simulink model "Copter_Plane_h2g_4_and_1"  (R2020a)
settings: Solver=ode1  StartTime=0.0  StopTime=100  FixedStep=dt  RelTol=1e-3
(part 1 of 2)
settings Model: xpc_rtwmakecfg_data=_xpcnblib_  PauseTimes=2  Creator=a4327  LastModifiedBy=a4327
settings DataIOCC: ReturnWorkspaceOutputs=off
settings OptimizationCC: DefaultParameterBehavior=Inlined  UseDivisionForNetSlopeComputation=on  GainParamInheritBuiltInType=on  UseFloatMulNetSlope=on  InlineInvariantSignals=on  PassReuseOutputArgsAs=Individual arguments  ZeroExternalMemoryAtStartup=off  ZeroInternalMemoryAtStartup=off  NoFixptDivByZeroProtection=on  EfficientFloat2IntCast=on  LifeSpan=1  OptimizeBlockOrder=speed  DifferentSizesBufferReuse=on  EfficientTunableParamExpr=on
settings DebuggingCC: ParameterTunabilityLossMsg=error  ArithmeticOperatorsInVariantConditions=warning
settings HardwareCC: ProdBitPerPointer=32  ProdBitPerSizeT=32  ProdBitPerPtrDiffT=32  ProdLargestAtomicFloat=None  ProdWordSize=32  ProdLongLongMode=on  ProdHWDeviceType=Custom Processor->Custom Processor
settings SFSimCC: MATLABDynamicMemAlloc=off  CustomCodeUndefinedFunction=UseInterfaceOnly
settings RTWCC: SystemTargetFile=ert.tlc  TemplateMakefile=ert_default_tmf  GenerateReport=on  IncludeHyperlinkInReport=on  LaunchReport=on  GenerateTraceInfo=on  GenerateTraceReport=on  GenerateTraceReportSl=on  GenerateTraceReportSf=on  GenerateTraceReportEml=on  GenerateCodeMetricsReport=on
settings CodeAppCC: ForceParamTrailComments=on  IgnoreCustomStorageClasses=off  OperatorAnnotations=on  SimulinkDataObjDesc=on  SFDataObjDesc=on  CustomSymbolStrGlobalVar=rt$N$M  CustomSymbolStrType=$N$M  CustomSymbolStrFcn=$N$M$F  CustomSymbolStrMacro=$N$M  InsertBlockDesc=on
settings ERTTargetCC: TargetLangStandard=C99 (ISO)  GenerateSampleERTMain=on  IncludeMdlTerminateFcn=off  CombineSignalStateStructs=on  MultiInstanceERTCode=on  CodeInterfacePackaging=Reusable function  SupportComplex=off  SupportNonInlinedSFcns=on  InlinedParameterPlacement=NonHierarchical  RootIOFormat=Structure reference  ERTCustomFileTemplate=example_file_process.tlc  ERTFilePackagingFormat=CompactWithDataFile

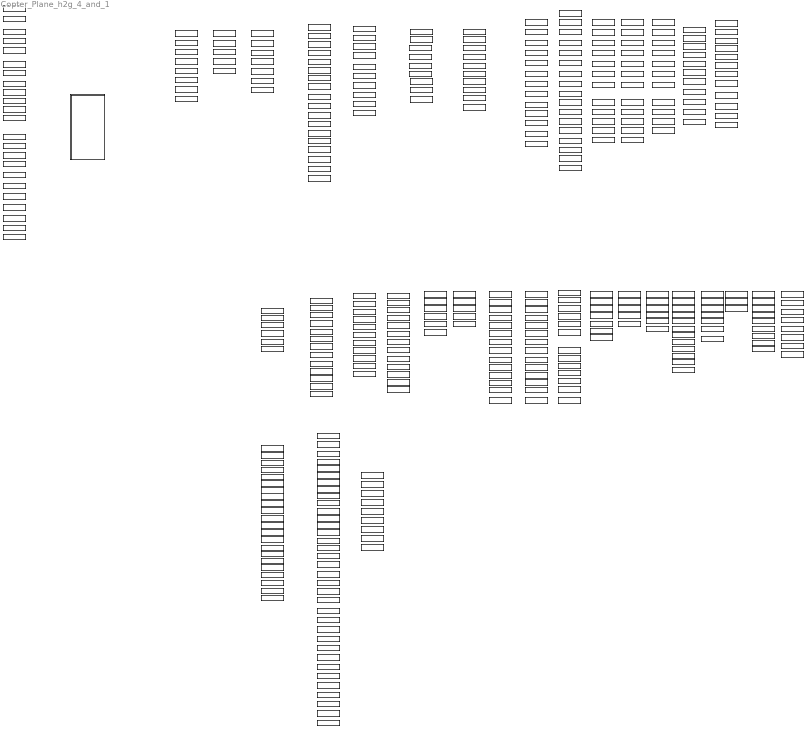
== system Copter_Plane_h2g_4_and_1 ==
  AC_ATTITUDE_ACCEL_RP_CONTROLLER_MAX_RADSS1 : DataStoreMemory  DataStoreName=AC_ATTITUDE_ACCEL_RP_CONTROLLER_MAX_RADSS  ReadBeforeWriteMsg=warning  WriteAfterWriteMsg=warning  WriteAfterReadMsg=warning  InitialValue=AC_ATTITUDE_ACCEL_RP_CONTROLLER_MAX_RADSS  VectorParams1D=off  ShowAdditionalParam=off  OutDataTypeStr=double
  AC_ATTITUDE_ACCEL_RP_CONTROLLER_MIN_RADSS1 : DataStoreMemory  DataStoreName=AC_ATTITUDE_ACCEL_RP_CONTROLLER_MIN_RADSS  ReadBeforeWriteMsg=warning  WriteAfterWriteMsg=warning  WriteAfterReadMsg=warning  InitialValue=AC_ATTITUDE_ACCEL_RP_CONTROLLER_MIN_RADSS  VectorParams1D=off  ShowAdditionalParam=off  OutDataTypeStr=double
  AC_ATTITUDE_ACCEL_Y_CONTROLLER_MAX_RADSS1 : DataStoreMemory  DataStoreName=AC_ATTITUDE_ACCEL_Y_CONTROLLER_MAX_RADSS  ReadBeforeWriteMsg=warning  WriteAfterWriteMsg=warning  WriteAfterReadMsg=warning  InitialValue=AC_ATTITUDE_ACCEL_Y_CONTROLLER_MAX_RADSS  ShowAdditionalParam=off  OutDataTypeStr=double
  AC_ATTITUDE_ACCEL_Y_CONTROLLER_MIN_RADSS1 : DataStoreMemory  DataStoreName=AC_ATTITUDE_ACCEL_Y_CONTROLLER_MIN_RADSS  ReadBeforeWriteMsg=warning  WriteAfterWriteMsg=warning  WriteAfterReadMsg=warning  InitialValue=AC_ATTITUDE_ACCEL_Y_CONTROLLER_MIN_RADSS  VectorParams1D=off  ShowAdditionalParam=off  OutDataTypeStr=double
  AC_ATTITUDE_CONTROL_ANGLE_LIMIT_THROTTLE_MAX1 : DataStoreMemory  DataStoreName=AC_ATTITUDE_CONTROL_ANGLE_LIMIT_THROTTLE_MAX  ReadBeforeWriteMsg=warning  WriteAfterWriteMsg=warning  WriteAfterReadMsg=warning  InitialValue=AC_ATTITUDE_CONTROL_ANGLE_LIMIT_THROTTLE_MAX  VectorParams1D=off  ShowAdditionalParam=off  OutDataTypeStr=double
  AC_ATTITUDE_CONTROL_MAX1 : DataStoreMemory  DataStoreName=AC_ATTITUDE_CONTROL_MAX  ReadBeforeWriteMsg=warning  WriteAfterWriteMsg=warning  WriteAfterReadMsg=warning  InitialValue=AC_ATTITUDE_CONTROL_MAX  VectorParams1D=off  ShowAdditionalParam=off  OutDataTypeStr=double
  AC_ATTITUDE_THRUST_ERROR_ANGLE1 : DataStoreMemory  DataStoreName=AC_ATTITUDE_THRUST_ERROR_ANGLE  ReadBeforeWriteMsg=warning  WriteAfterWriteMsg=warning  WriteAfterReadMsg=warning  InitialValue=AC_ATTITUDE_THRUST_ERROR_ANGLE  ShowAdditionalParam=off  OutDataTypeStr=double
  AP_MOTORS_MATRIX_YAW_FACTOR_CCW1 : DataStoreMemory  DataStoreName=AP_MOTORS_MATRIX_YAW_FACTOR_CCW  ReadBeforeWriteMsg=warning  WriteAfterWriteMsg=warning  WriteAfterReadMsg=warning  InitialValue=AP_MOTORS_MATRIX_YAW_FACTOR_CCW  VectorParams1D=off  ShowAdditionalParam=off  OutDataTypeStr=double
  AP_MOTORS_MATRIX_YAW_FACTOR_CW1 : DataStoreMemory  DataStoreName=AP_MOTORS_MATRIX_YAW_FACTOR_CW  ReadBeforeWriteMsg=warning  WriteAfterWriteMsg=warning  WriteAfterReadMsg=warning  InitialValue=AP_MOTORS_MATRIX_YAW_FACTOR_CW  VectorParams1D=off  ShowAdditionalParam=off  OutDataTypeStr=double
  ATC_RAT_PIT_D1 : DataStoreMemory  DataStoreName=ATC_RAT_PIT_D  ReadBeforeWriteMsg=warning  WriteAfterWriteMsg=warning  WriteAfterReadMsg=warning  InitialValue=ATC_RAT_PIT_D  VectorParams1D=off  ShowAdditionalParam=off  OutDataTypeStr=double
  ATC_RAT_PIT_FF1 : DataStoreMemory  DataStoreName=ATC_RAT_PIT_FF  ReadBeforeWriteMsg=warning  WriteAfterWriteMsg=warning  WriteAfterReadMsg=warning  InitialValue=ATC_RAT_PIT_FF  VectorParams1D=off  ShowAdditionalParam=off  OutDataTypeStr=double
  ATC_RAT_PIT_FILT1 : DataStoreMemory  DataStoreName=ATC_RAT_PIT_FILT  ReadBeforeWriteMsg=warning  WriteAfterWriteMsg=warning  WriteAfterReadMsg=warning  InitialValue=ATC_RAT_PIT_FILT  VectorParams1D=off  ShowAdditionalParam=off  OutDataTypeStr=double
  ATC_RAT_PIT_I1 : DataStoreMemory  DataStoreName=ATC_RAT_PIT_I  ReadBeforeWriteMsg=warning  WriteAfterWriteMsg=warning  WriteAfterReadMsg=warning  InitialValue=ATC_RAT_PIT_I  VectorParams1D=off  ShowAdditionalParam=off  OutDataTypeStr=double
  ATC_RAT_PIT_IMAX1 : DataStoreMemory  DataStoreName=ATC_RAT_PIT_IMAX  ReadBeforeWriteMsg=warning  WriteAfterWriteMsg=warning  WriteAfterReadMsg=warning  InitialValue=ATC_RAT_PIT_IMAX  VectorParams1D=off  ShowAdditionalParam=off  OutDataTypeStr=double
  ATC_RAT_PIT_I_inint1 : DataStoreMemory  DataStoreName=ATC_RAT_PIT_I_inint  ReadBeforeWriteMsg=warning  WriteAfterWriteMsg=warning  WriteAfterReadMsg=warning  InitialValue=ATC_RAT_PIT_I_inint  VectorParams1D=off  ShowAdditionalParam=off  OutDataTypeStr=double
  ATC_RAT_PIT_P1 : DataStoreMemory  DataStoreName=ATC_RAT_PIT_P  ReadBeforeWriteMsg=warning  WriteAfterWriteMsg=warning  WriteAfterReadMsg=warning  InitialValue=ATC_RAT_PIT_P  VectorParams1D=off  ShowAdditionalParam=off  OutDataTypeStr=double
  ATC_RAT_RLL_D1 : DataStoreMemory  DataStoreName=ATC_RAT_RLL_D  ReadBeforeWriteMsg=warning  WriteAfterWriteMsg=warning  WriteAfterReadMsg=warning  InitialValue=ATC_RAT_RLL_D  VectorParams1D=off  ShowAdditionalParam=off  OutDataTypeStr=double
  ATC_RAT_RLL_FF1 : DataStoreMemory  DataStoreName=ATC_RAT_RLL_FF  ReadBeforeWriteMsg=warning  WriteAfterWriteMsg=warning  WriteAfterReadMsg=warning  InitialValue=ATC_RAT_RLL_FF  VectorParams1D=off  ShowAdditionalParam=off  OutDataTypeStr=double
  ATC_RAT_RLL_FILT1 : DataStoreMemory  DataStoreName=ATC_RAT_RLL_FILT  ReadBeforeWriteMsg=warning  WriteAfterWriteMsg=warning  WriteAfterReadMsg=warning  InitialValue=ATC_RAT_RLL_FILT  VectorParams1D=off  ShowAdditionalParam=off  OutDataTypeStr=double
  ATC_RAT_RLL_I1 : DataStoreMemory  DataStoreName=ATC_RAT_RLL_I  ReadBeforeWriteMsg=warning  WriteAfterWriteMsg=warning  WriteAfterReadMsg=warning  InitialValue=ATC_RAT_RLL_I  VectorParams1D=off  ShowAdditionalParam=off  OutDataTypeStr=double
  ATC_RAT_RLL_IMAX1 : DataStoreMemory  DataStoreName=ATC_RAT_RLL_IMAX  ReadBeforeWriteMsg=warning  WriteAfterWriteMsg=warning  WriteAfterReadMsg=warning  InitialValue=ATC_RAT_RLL_IMAX  VectorParams1D=off  ShowAdditionalParam=off  OutDataTypeStr=double
  ATC_RAT_RLL_I_inint1 : DataStoreMemory  DataStoreName=ATC_RAT_RLL_I_inint  ReadBeforeWriteMsg=warning  WriteAfterWriteMsg=warning  WriteAfterReadMsg=warning  InitialValue=ATC_RAT_RLL_I_inint  VectorParams1D=off  ShowAdditionalParam=off  OutDataTypeStr=double
  ATC_RAT_RLL_P1 : DataStoreMemory  DataStoreName=ATC_RAT_RLL_P  ReadBeforeWriteMsg=warning  WriteAfterWriteMsg=warning  WriteAfterReadMsg=warning  InitialValue=ATC_RAT_RLL_P  VectorParams1D=off  ShowAdditionalParam=off  OutDataTypeStr=double
  ATC_RAT_YAW_D1 : DataStoreMemory  DataStoreName=ATC_RAT_YAW_D  ReadBeforeWriteMsg=warning  WriteAfterWriteMsg=warning  WriteAfterReadMsg=warning  InitialValue=ATC_RAT_YAW_D  VectorParams1D=off  ShowAdditionalParam=off  OutDataTypeStr=double
  ATC_RAT_YAW_FF1 : DataStoreMemory  DataStoreName=ATC_RAT_YAW_FF  ReadBeforeWriteMsg=warning  WriteAfterWriteMsg=warning  WriteAfterReadMsg=warning  InitialValue=ATC_RAT_YAW_FF  VectorParams1D=off  ShowAdditionalParam=off  OutDataTypeStr=double
  ATC_RAT_YAW_FILT1 : DataStoreMemory  DataStoreName=ATC_RAT_YAW_FILT  ReadBeforeWriteMsg=warning  WriteAfterWriteMsg=warning  WriteAfterReadMsg=warning  InitialValue=ATC_RAT_YAW_FILT  VectorParams1D=off  ShowAdditionalParam=off  OutDataTypeStr=double
  ATC_RAT_YAW_I1 : DataStoreMemory  DataStoreName=ATC_RAT_YAW_I  ReadBeforeWriteMsg=warning  WriteAfterWriteMsg=warning  WriteAfterReadMsg=warning  InitialValue=ATC_RAT_YAW_I  VectorParams1D=off  ShowAdditionalParam=off  OutDataTypeStr=double
  ATC_RAT_YAW_IMAX1 : DataStoreMemory  DataStoreName=ATC_RAT_YAW_IMAX  ReadBeforeWriteMsg=warning  WriteAfterWriteMsg=warning  WriteAfterReadMsg=warning  InitialValue=ATC_RAT_YAW_IMAX  VectorParams1D=off  ShowAdditionalParam=off  OutDataTypeStr=double
  ATC_RAT_YAW_I_inint1 : DataStoreMemory  DataStoreName=ATC_RAT_YAW_I_inint  ReadBeforeWriteMsg=warning  WriteAfterWriteMsg=warning  WriteAfterReadMsg=warning  InitialValue=ATC_RAT_YAW_I_inint  VectorParams1D=off  ShowAdditionalParam=off  OutDataTypeStr=double
  ATC_RAT_YAW_P1 : DataStoreMemory  DataStoreName=ATC_RAT_YAW_P  ReadBeforeWriteMsg=warning  WriteAfterWriteMsg=warning  WriteAfterReadMsg=warning  InitialValue=ATC_RAT_YAW_P  VectorParams1D=off  ShowAdditionalParam=off  OutDataTypeStr=double
  EAS2TAS1 : DataStoreMemory  DataStoreName=EAS2TAS  ReadBeforeWriteMsg=warning  WriteAfterWriteMsg=warning  WriteAfterReadMsg=warning  InitialValue=EAS2TAS  VectorParams1D=off  ShowAdditionalParam=off  OutDataTypeStr=double
  EAS_dem1 : DataStoreMemory  DataStoreName=EAS_dem  ReadBeforeWriteMsg=warning  WriteAfterWriteMsg=warning  WriteAfterReadMsg=warning  InitialValue=EAS_dem  VectorParams1D=off  ShowAdditionalParam=off  OutDataTypeStr=double
  EAS_dem_cm1 : DataStoreMemory  DataStoreName=EAS_dem_cm  ReadBeforeWriteMsg=warning  WriteAfterWriteMsg=warning  WriteAfterReadMsg=warning  InitialValue=EAS_dem_cm  VectorParams1D=off  ShowAdditionalParam=off  OutDataTypeStr=double
  GRAVITY_MSS1 : DataStoreMemory  DataStoreName=GRAVITY_MSS  ReadBeforeWriteMsg=warning  WriteAfterWriteMsg=warning  WriteAfterReadMsg=warning  InitialValue=GRAVITY_MSS  VectorParams1D=off  ShowAdditionalParam=off  OutDataTypeStr=double
  HD1 : DataStoreMemory  DataStoreName=HD  ReadBeforeWriteMsg=warning  WriteAfterWriteMsg=warning  WriteAfterReadMsg=warning  InitialValue=HD  ShowAdditionalParam=off  OutDataTypeStr=double
  K_A_yaw1 : DataStoreMemory  DataStoreName=K_A_yaw  ReadBeforeWriteMsg=warning  WriteAfterWriteMsg=warning  WriteAfterReadMsg=warning  InitialValue=K_A_yaw  ShowAdditionalParam=off  OutDataTypeStr=double
  K_D_last_yaw1 : DataStoreMemory  DataStoreName=K_D_last_yaw  ReadBeforeWriteMsg=warning  WriteAfterWriteMsg=warning  WriteAfterReadMsg=warning  InitialValue=K_D_last_yaw  ShowAdditionalParam=off  OutDataTypeStr=double
  K_D_yaw1 : DataStoreMemory  DataStoreName=K_D_yaw  ReadBeforeWriteMsg=warning  WriteAfterWriteMsg=warning  WriteAfterReadMsg=warning  InitialValue=K_D_yaw  ShowAdditionalParam=off  OutDataTypeStr=double
  K_FF_yaw1 : DataStoreMemory  DataStoreName=K_FF_yaw  ReadBeforeWriteMsg=warning  WriteAfterWriteMsg=warning  WriteAfterReadMsg=warning  InitialValue=K_FF_yaw  ShowAdditionalParam=off  OutDataTypeStr=double
  K_FF_yaw_inint1 : DataStoreMemory  DataStoreName=K_FF_yaw_inint  ReadBeforeWriteMsg=warning  WriteAfterWriteMsg=warning  WriteAfterReadMsg=warning  InitialValue=K_FF_yaw_inint  VectorParams1D=off  ShowAdditionalParam=off  OutDataTypeStr=double
  K_I_yaw1 : DataStoreMemory  DataStoreName=K_I_yaw  ReadBeforeWriteMsg=warning  WriteAfterWriteMsg=warning  WriteAfterReadMsg=warning  InitialValue=K_I_yaw  ShowAdditionalParam=off  OutDataTypeStr=double
  Kx1 : DataStoreMemory  DataStoreName=Kx  ReadBeforeWriteMsg=warning  WriteAfterWriteMsg=warning  WriteAfterReadMsg=warning  InitialValue=Kx  VectorParams1D=off  ShowAdditionalParam=off  OutDataTypeStr=double
  L1_damping1 : DataStoreMemory  DataStoreName=L1_damping  ReadBeforeWriteMsg=warning  WriteAfterWriteMsg=warning  WriteAfterReadMsg=warning  InitialValue=L1_damping  VectorParams1D=off  ShowAdditionalParam=off  OutDataTypeStr=double
  L1_dist1 : DataStoreMemory  DataStoreName=L1_dist  ReadBeforeWriteMsg=warning  WriteAfterWriteMsg=warning  WriteAfterReadMsg=warning  InitialValue=L1_dist  VectorParams1D=off  ShowAdditionalParam=off  OutDataTypeStr=double
  L1_period1 : DataStoreMemory  DataStoreName=L1_period  ReadBeforeWriteMsg=warning  WriteAfterWriteMsg=warning  WriteAfterReadMsg=warning  InitialValue=L1_period  VectorParams1D=off  ShowAdditionalParam=off  OutDataTypeStr=double
  L1_radius1 : DataStoreMemory  DataStoreName=L1_radius  ReadBeforeWriteMsg=warning  WriteAfterWriteMsg=warning  WriteAfterReadMsg=warning  InitialValue=L1_radius  VectorParams1D=off  ShowAdditionalParam=off  OutDataTypeStr=double
  L1_xtrack_i1 : DataStoreMemory  DataStoreName=L1_xtrack_i  ReadBeforeWriteMsg=warning  WriteAfterWriteMsg=warning  WriteAfterReadMsg=warning  InitialValue=L1_xtrack_i  VectorParams1D=off  ShowAdditionalParam=off  OutDataTypeStr=double
  L1_xtrack_i_gain1 : DataStoreMemory  DataStoreName=L1_xtrack_i_gain  ReadBeforeWriteMsg=warning  WriteAfterWriteMsg=warning  WriteAfterReadMsg=warning  InitialValue=L1_xtrack_i_gain  VectorParams1D=off  ShowAdditionalParam=off  OutDataTypeStr=double
  L1_xtrack_i_gain_prev1 : DataStoreMemory  DataStoreName=L1_xtrack_i_gain_prev  ReadBeforeWriteMsg=warning  WriteAfterWriteMsg=warning  WriteAfterReadMsg=warning  InitialValue=L1_xtrack_i_gain_prev  VectorParams1D=off  ShowAdditionalParam=off  OutDataTypeStr=double
  LOCATION_SCALING_FACTOR1 : DataStoreMemory  DataStoreName=LOCATION_SCALING_FACTOR  ReadBeforeWriteMsg=warning  WriteAfterWriteMsg=warning  WriteAfterReadMsg=warning  InitialValue=LOCATION_SCALING_FACTOR  VectorParams1D=off  ShowAdditionalParam=off  OutDataTypeStr=double
  LOCATION_SCALING_FACTOR_INV1 : DataStoreMemory  DataStoreName=LOCATION_SCALING_FACTOR_INV  ReadBeforeWriteMsg=warning  WriteAfterWriteMsg=warning  WriteAfterReadMsg=warning  InitialValue=LOCATION_SCALING_FACTOR_INV  VectorParams1D=off  ShowAdditionalParam=off  OutDataTypeStr=double
  PITCHmaxf1 : DataStoreMemory  DataStoreName=PITCHmaxf  ReadBeforeWriteMsg=warning  WriteAfterWriteMsg=warning  WriteAfterReadMsg=warning  InitialValue=PITCHmaxf  VectorParams1D=off  ShowAdditionalParam=off  OutDataTypeStr=double
  PITCHminf1 : DataStoreMemory  DataStoreName=PITCHminf  ReadBeforeWriteMsg=warning  WriteAfterWriteMsg=warning  WriteAfterReadMsg=warning  InitialValue=PITCHminf  VectorParams1D=off  ShowAdditionalParam=off  OutDataTypeStr=double
  POSCONTROL_ACCELERATION_MIN1 : DataStoreMemory  DataStoreName=POSCONTROL_ACCELERATION_MIN  ReadBeforeWriteMsg=warning  WriteAfterWriteMsg=warning  WriteAfterReadMsg=warning  InitialValue=POSCONTROL_ACCELERATION_MIN  ShowAdditionalParam=off  OutDataTypeStr=double
  POSCONTROL_ACCEL_FILTER_HZ1 : DataStoreMemory  DataStoreName=POSCONTROL_ACCEL_FILTER_HZ  ReadBeforeWriteMsg=warning  WriteAfterWriteMsg=warning  WriteAfterReadMsg=warning  InitialValue=POSCONTROL_ACCEL_FILTER_HZ  VectorParams1D=off  ShowAdditionalParam=off  OutDataTypeStr=double
  POSCONTROL_ACCEL_XY1 : DataStoreMemory  DataStoreName=POSCONTROL_ACCEL_XY  ReadBeforeWriteMsg=warning  WriteAfterWriteMsg=warning  WriteAfterReadMsg=warning  InitialValue=POSCONTROL_ACCEL_XY  VectorParams1D=off  ShowAdditionalParam=off  OutDataTypeStr=double
  POSCONTROL_ACCEL_XY_MAX1 : DataStoreMemory  DataStoreName=POSCONTROL_ACCEL_XY_MAX  ReadBeforeWriteMsg=warning  WriteAfterWriteMsg=warning  WriteAfterReadMsg=warning  InitialValue=POSCONTROL_ACCEL_XY_MAX  VectorParams1D=off  ShowAdditionalParam=off  OutDataTypeStr=double
  POSCONTROL_ACCEL_Z1 : DataStoreMemory  DataStoreName=POSCONTROL_ACCEL_Z  ReadBeforeWriteMsg=warning  WriteAfterWriteMsg=warning  WriteAfterReadMsg=warning  InitialValue=POSCONTROL_ACCEL_Z  ShowAdditionalParam=off  OutDataTypeStr=double
  POSCONTROL_ACC_Z_D1 : DataStoreMemory  DataStoreName=POSCONTROL_ACC_Z_D  ReadBeforeWriteMsg=warning  WriteAfterWriteMsg=warning  WriteAfterReadMsg=warning  InitialValue=POSCONTROL_ACC_Z_D  VectorParams1D=off  ShowAdditionalParam=off  OutDataTypeStr=double
  POSCONTROL_ACC_Z_FILT_HZ1 : DataStoreMemory  DataStoreName=POSCONTROL_ACC_Z_FILT_HZ  ReadBeforeWriteMsg=warning  WriteAfterWriteMsg=warning  WriteAfterReadMsg=warning  InitialValue=POSCONTROL_ACC_Z_FILT_HZ  VectorParams1D=off  ShowAdditionalParam=off  OutDataTypeStr=double
  POSCONTROL_ACC_Z_FILT_HZ_c2p1 : DataStoreMemory  DataStoreName=POSCONTROL_ACC_Z_FILT_HZ_c2p  ReadBeforeWriteMsg=warning  WriteAfterWriteMsg=warning  WriteAfterReadMsg=warning  InitialValue=POSCONTROL_ACC_Z_FILT_HZ_c2p  VectorParams1D=off  ShowAdditionalParam=off  OutDataTypeStr=double
  POSCONTROL_ACC_Z_FILT_HZ_inint1 : DataStoreMemory  DataStoreName=POSCONTROL_ACC_Z_FILT_HZ_inint  ReadBeforeWriteMsg=warning  WriteAfterWriteMsg=warning  WriteAfterReadMsg=warning  InitialValue=POSCONTROL_ACC_Z_FILT_HZ_inint  VectorParams1D=off  ShowAdditionalParam=off  OutDataTypeStr=double
  POSCONTROL_ACC_Z_I1 : DataStoreMemory  DataStoreName=POSCONTROL_ACC_Z_I  ReadBeforeWriteMsg=warning  WriteAfterWriteMsg=warning  WriteAfterReadMsg=warning  InitialValue=POSCONTROL_ACC_Z_I  VectorParams1D=off  ShowAdditionalParam=off  OutDataTypeStr=double
  POSCONTROL_ACC_Z_IMAX1 : DataStoreMemory  DataStoreName=POSCONTROL_ACC_Z_IMAX  ReadBeforeWriteMsg=warning  WriteAfterWriteMsg=warning  WriteAfterReadMsg=warning  InitialValue=POSCONTROL_ACC_Z_IMAX  VectorParams1D=off  ShowAdditionalParam=off  OutDataTypeStr=double
  POSCONTROL_ACC_Z_I_inint1 : DataStoreMemory  DataStoreName=POSCONTROL_ACC_Z_I_inint  ReadBeforeWriteMsg=warning  WriteAfterWriteMsg=warning  WriteAfterReadMsg=warning  InitialValue=POSCONTROL_ACC_Z_I_inint  VectorParams1D=off  ShowAdditionalParam=off  OutDataTypeStr=double
  POSCONTROL_ACC_Z_P1 : DataStoreMemory  DataStoreName=POSCONTROL_ACC_Z_P  ReadBeforeWriteMsg=warning  WriteAfterWriteMsg=warning  WriteAfterReadMsg=warning  InitialValue=POSCONTROL_ACC_Z_P  VectorParams1D=off  ShowAdditionalParam=off  OutDataTypeStr=double
  POSCONTROL_JERK_RATIO1 : DataStoreMemory  DataStoreName=POSCONTROL_JERK_RATIO  ReadBeforeWriteMsg=warning  WriteAfterWriteMsg=warning  WriteAfterReadMsg=warning  InitialValue=POSCONTROL_JERK_RATIO  VectorParams1D=off  ShowAdditionalParam=off  OutDataTypeStr=double
  POSCONTROL_LEASH_LENGTH_MIN1 : DataStoreMemory  DataStoreName=POSCONTROL_LEASH_LENGTH_MIN  ReadBeforeWriteMsg=warning  WriteAfterWriteMsg=warning  WriteAfterReadMsg=warning  InitialValue=POSCONTROL_LEASH_LENGTH_MIN  VectorParams1D=off  ShowAdditionalParam=off  OutDataTypeStr=double
  POSCONTROL_OVERSPEED_GAIN_Z1 : DataStoreMemory  DataStoreName=POSCONTROL_OVERSPEED_GAIN_Z  ReadBeforeWriteMsg=warning  WriteAfterWriteMsg=warning  WriteAfterReadMsg=warning  InitialValue=POSCONTROL_OVERSPEED_GAIN_Z  VectorParams1D=off  ShowAdditionalParam=off  OutDataTypeStr=double
  POSCONTROL_POS_XY_P1 : DataStoreMemory  DataStoreName=POSCONTROL_POS_XY_P  ReadBeforeWriteMsg=warning  WriteAfterWriteMsg=warning  WriteAfterReadMsg=warning  InitialValue=POSCONTROL_POS_XY_P  VectorParams1D=off  ShowAdditionalParam=off  OutDataTypeStr=double
  POSCONTROL_POS_Z_P1 : DataStoreMemory  DataStoreName=POSCONTROL_POS_Z_P  ReadBeforeWriteMsg=warning  WriteAfterWriteMsg=warning  WriteAfterReadMsg=warning  InitialValue=POSCONTROL_POS_Z_P  VectorParams1D=off  ShowAdditionalParam=off  OutDataTypeStr=double
  POSCONTROL_SPEED1 : DataStoreMemory  DataStoreName=POSCONTROL_SPEED  ReadBeforeWriteMsg=warning  WriteAfterWriteMsg=warning  WriteAfterReadMsg=warning  InitialValue=POSCONTROL_SPEED  ShowAdditionalParam=off  OutDataTypeStr=double
  POSCONTROL_SPEED_DOWN1 : DataStoreMemory  DataStoreName=POSCONTROL_SPEED_DOWN  ReadBeforeWriteMsg=warning  WriteAfterWriteMsg=warning  WriteAfterReadMsg=warning  InitialValue=POSCONTROL_SPEED_DOWN  ShowAdditionalParam=off  OutDataTypeStr=double
  POSCONTROL_SPEED_UP1 : DataStoreMemory  DataStoreName=POSCONTROL_SPEED_UP  ReadBeforeWriteMsg=warning  WriteAfterWriteMsg=warning  WriteAfterReadMsg=warning  InitialValue=POSCONTROL_SPEED_UP  ShowAdditionalParam=off  OutDataTypeStr=double
  POSCONTROL_STOPPING_DIST_DOWN_MAX1 : DataStoreMemory  DataStoreName=POSCONTROL_STOPPING_DIST_DOWN_MAX  ReadBeforeWriteMsg=warning  WriteAfterWriteMsg=warning  WriteAfterReadMsg=warning  InitialValue=POSCONTROL_STOPPING_DIST_DOWN_MAX  VectorParams1D=off  ShowAdditionalParam=off  OutDataTypeStr=double
  POSCONTROL_STOPPING_DIST_UP_MAX1 : DataStoreMemory  DataStoreName=POSCONTROL_STOPPING_DIST_UP_MAX  ReadBeforeWriteMsg=warning  WriteAfterWriteMsg=warning  WriteAfterReadMsg=warning  InitialValue=POSCONTROL_STOPPING_DIST_UP_MAX  VectorParams1D=off  ShowAdditionalParam=off  OutDataTypeStr=double
  POSCONTROL_THROTTLE_CUTOFF_FREQ1 : DataStoreMemory  DataStoreName=POSCONTROL_THROTTLE_CUTOFF_FREQ  ReadBeforeWriteMsg=warning  WriteAfterWriteMsg=warning  WriteAfterReadMsg=warning  InitialValue=POSCONTROL_THROTTLE_CUTOFF_FREQ  VectorParams1D=off  ShowAdditionalParam=off  OutDataTypeStr=double
  POSCONTROL_VEL_ERROR_CUTOFF_FREQ1 : DataStoreMemory  DataStoreName=POSCONTROL_VEL_ERROR_CUTOFF_FREQ  ReadBeforeWriteMsg=warning  WriteAfterWriteMsg=warning  WriteAfterReadMsg=warning  InitialValue=POSCONTROL_VEL_ERROR_CUTOFF_FREQ  VectorParams1D=off  ShowAdditionalParam=off  OutDataTypeStr=double
  POSCONTROL_VEL_XY_D1 : DataStoreMemory  DataStoreName=POSCONTROL_VEL_XY_D  ReadBeforeWriteMsg=warning  WriteAfterWriteMsg=warning  WriteAfterReadMsg=warning  InitialValue=POSCONTROL_VEL_XY_D  VectorParams1D=off  ShowAdditionalParam=off  OutDataTypeStr=double
  POSCONTROL_VEL_XY_FILT_D_HZ1 : DataStoreMemory  DataStoreName=POSCONTROL_VEL_XY_FILT_D_HZ  ReadBeforeWriteMsg=warning  WriteAfterWriteMsg=warning  WriteAfterReadMsg=warning  InitialValue=POSCONTROL_VEL_XY_FILT_D_HZ  VectorParams1D=off  ShowAdditionalParam=off  OutDataTypeStr=double
  POSCONTROL_VEL_XY_FILT_HZ1 : DataStoreMemory  DataStoreName=POSCONTROL_VEL_XY_FILT_HZ  ReadBeforeWriteMsg=warning  WriteAfterWriteMsg=warning  WriteAfterReadMsg=warning  InitialValue=POSCONTROL_VEL_XY_FILT_HZ  VectorParams1D=off  ShowAdditionalParam=off  OutDataTypeStr=double
  POSCONTROL_VEL_XY_I1 : DataStoreMemory  DataStoreName=POSCONTROL_VEL_XY_I  ReadBeforeWriteMsg=warning  WriteAfterWriteMsg=warning  WriteAfterReadMsg=warning  InitialValue=POSCONTROL_VEL_XY_I  VectorParams1D=off  ShowAdditionalParam=off  OutDataTypeStr=double
  POSCONTROL_VEL_XY_IMAX1 : DataStoreMemory  DataStoreName=POSCONTROL_VEL_XY_IMAX  ReadBeforeWriteMsg=warning  WriteAfterWriteMsg=warning  WriteAfterReadMsg=warning  InitialValue=POSCONTROL_VEL_XY_IMAX  VectorParams1D=off  ShowAdditionalParam=off  OutDataTypeStr=double
  POSCONTROL_VEL_XY_I_inint1 : DataStoreMemory  DataStoreName=POSCONTROL_VEL_XY_I_inint  ReadBeforeWriteMsg=warning  WriteAfterWriteMsg=warning  WriteAfterReadMsg=warning  InitialValue=POSCONTROL_VEL_XY_I_inint  VectorParams1D=off  ShowAdditionalParam=off  OutDataTypeStr=double
  POSCONTROL_VEL_XY_P1 : DataStoreMemory  DataStoreName=POSCONTROL_VEL_XY_P  ReadBeforeWriteMsg=warning  WriteAfterWriteMsg=warning  WriteAfterReadMsg=warning  InitialValue=POSCONTROL_VEL_XY_P  VectorParams1D=off  ShowAdditionalParam=off  OutDataTypeStr=double
  POSCONTROL_VEL_Z_P1 : DataStoreMemory  DataStoreName=POSCONTROL_VEL_Z_P  ReadBeforeWriteMsg=warning  WriteAfterWriteMsg=warning  WriteAfterReadMsg=warning  InitialValue=POSCONTROL_VEL_Z_P  VectorParams1D=off  ShowAdditionalParam=off  OutDataTypeStr=double
  PathModeOut1 : DataStoreMemory  DataStoreName=PathModeOut_sl  ReadBeforeWriteMsg=warning  WriteAfterWriteMsg=warning  WriteAfterReadMsg=warning  InitialValue=PathModeOut_sl  VectorParams1D=off  ShowAdditionalParam=off  OutDataTypeStr=Bus: BUS_TASK_PATH_OutParam
  SKE_dem1 : DataStoreMemory  DataStoreName=SKE_dem  ReadBeforeWriteMsg=warning  WriteAfterWriteMsg=warning  WriteAfterReadMsg=warning  InitialValue=SKE_dem  VectorParams1D=off  ShowAdditionalParam=off  OutDataTypeStr=double
  SKE_est1 : DataStoreMemory  DataStoreName=SKE_est  ReadBeforeWriteMsg=warning  WriteAfterWriteMsg=warning  WriteAfterReadMsg=warning  InitialValue=SKE_est  VectorParams1D=off  ShowAdditionalParam=off  OutDataTypeStr=double
  SKEdot1 : DataStoreMemory  DataStoreName=SKEdot  ReadBeforeWriteMsg=warning  WriteAfterWriteMsg=warning  WriteAfterReadMsg=warning  InitialValue=SKEdot  VectorParams1D=off  ShowAdditionalParam=off  OutDataTypeStr=double
  SKEdot_dem1 : DataStoreMemory  DataStoreName=SKEdot_dem  ReadBeforeWriteMsg=warning  WriteAfterWriteMsg=warning  WriteAfterReadMsg=warning  InitialValue=SKEdot_dem  VectorParams1D=off  ShowAdditionalParam=off  OutDataTypeStr=double
  SPE_dem1 : DataStoreMemory  DataStoreName=SPE_dem  ReadBeforeWriteMsg=warning  WriteAfterWriteMsg=warning  WriteAfterReadMsg=warning  InitialValue=SPE_dem  VectorParams1D=off  ShowAdditionalParam=off  OutDataTypeStr=double
  SPE_est1 : DataStoreMemory  DataStoreName=SPE_est  ReadBeforeWriteMsg=warning  WriteAfterWriteMsg=warning  WriteAfterReadMsg=warning  InitialValue=SPE_est  VectorParams1D=off  ShowAdditionalParam=off  OutDataTypeStr=double
  SPEdot1 : DataStoreMemory  DataStoreName=SPEdot  ReadBeforeWriteMsg=warning  WriteAfterWriteMsg=warning  WriteAfterReadMsg=warning  InitialValue=SPEdot  VectorParams1D=off  ShowAdditionalParam=off  OutDataTypeStr=double
  SPEdot_dem1 : DataStoreMemory  DataStoreName=SPEdot_dem  ReadBeforeWriteMsg=warning  WriteAfterWriteMsg=warning  WriteAfterReadMsg=warning  InitialValue=SPEdot_dem  VectorParams1D=off  ShowAdditionalParam=off  OutDataTypeStr=double
  STE_error1 : DataStoreMemory  DataStoreName=STE_error  ReadBeforeWriteMsg=warning  WriteAfterWriteMsg=warning  WriteAfterReadMsg=warning  InitialValue=STE_error  VectorParams1D=off  ShowAdditionalParam=off  OutDataTypeStr=double
  STEdotErrLast1 : DataStoreMemory  DataStoreName=STEdotErrLast  ReadBeforeWriteMsg=warning  WriteAfterWriteMsg=warning  WriteAfterReadMsg=warning  InitialValue=STEdotErrLast  VectorParams1D=off  ShowAdditionalParam=off  OutDataTypeStr=double
  STEdot_max1 : DataStoreMemory  DataStoreName=STEdot_max  ReadBeforeWriteMsg=warning  WriteAfterWriteMsg=warning  WriteAfterReadMsg=warning  InitialValue=STEdot_max  VectorParams1D=off  ShowAdditionalParam=off  OutDataTypeStr=double
  STEdot_min1 : DataStoreMemory  DataStoreName=STEdot_min  ReadBeforeWriteMsg=warning  WriteAfterWriteMsg=warning  WriteAfterReadMsg=warning  InitialValue=STEdot_min  VectorParams1D=off  ShowAdditionalParam=off  OutDataTypeStr=double
  TAS_dem1 : DataStoreMemory  DataStoreName=TAS_dem  ReadBeforeWriteMsg=warning  WriteAfterWriteMsg=warning  WriteAfterReadMsg=warning  InitialValue=TAS_dem  VectorParams1D=off  ShowAdditionalParam=off  OutDataTypeStr=double
  TAS_dem_adj1 : DataStoreMemory  DataStoreName=TAS_dem_adj  ReadBeforeWriteMsg=warning  WriteAfterWriteMsg=warning  WriteAfterReadMsg=warning  InitialValue=TAS_dem_adj  VectorParams1D=off  ShowAdditionalParam=off  OutDataTypeStr=double
  TAS_rate_dem1 : DataStoreMemory  DataStoreName=TAS_rate_dem  ReadBeforeWriteMsg=warning  WriteAfterWriteMsg=warning  WriteAfterReadMsg=warning  InitialValue=TAS_rate_dem  VectorParams1D=off  ShowAdditionalParam=off  OutDataTypeStr=double
  TAS_state1 : DataStoreMemory  DataStoreName=TAS_state  ReadBeforeWriteMsg=warning  WriteAfterWriteMsg=warning  WriteAfterReadMsg=warning  InitialValue=TAS_state  VectorParams1D=off  ShowAdditionalParam=off  OutDataTypeStr=double
  TASmax1 : DataStoreMemory  DataStoreName=TASmax  ReadBeforeWriteMsg=warning  WriteAfterWriteMsg=warning  WriteAfterReadMsg=warning  InitialValue=TASmax  VectorParams1D=off  ShowAdditionalParam=off  OutDataTypeStr=double
  TASmin1 : DataStoreMemory  DataStoreName=TASmin  ReadBeforeWriteMsg=warning  WriteAfterWriteMsg=warning  WriteAfterReadMsg=warning  InitialValue=TASmin  VectorParams1D=off  ShowAdditionalParam=off  OutDataTypeStr=double
  THRmaxf1 : DataStoreMemory  DataStoreName=THRmaxf  ReadBeforeWriteMsg=warning  WriteAfterWriteMsg=warning  WriteAfterReadMsg=warning  InitialValue=THRmaxf  VectorParams1D=off  ShowAdditionalParam=off  OutDataTypeStr=double
  THRminf1 : DataStoreMemory  DataStoreName=THRminf  ReadBeforeWriteMsg=warning  WriteAfterWriteMsg=warning  WriteAfterReadMsg=warning  InitialValue=THRminf  VectorParams1D=off  ShowAdditionalParam=off  OutDataTypeStr=double
  Vz1 : DataStoreMemory  DataStoreName=Vz  ReadBeforeWriteMsg=warning  WriteAfterWriteMsg=warning  WriteAfterReadMsg=warning  InitialValue=Vz  ShowAdditionalParam=off  OutDataTypeStr=double
  WPcircle1 : DataStoreMemory  DataStoreName=WPcircle  ReadBeforeWriteMsg=warning  WriteAfterWriteMsg=warning  WriteAfterReadMsg=warning  InitialValue=WPcircle  VectorParams1D=off  ShowAdditionalParam=off  OutDataTypeStr=double
  accel_desired1 : DataStoreMemory  DataStoreName=accel_desired  ReadBeforeWriteMsg=warning  WriteAfterWriteMsg=warning  WriteAfterReadMsg=warning  InitialValue=accel_desired  VectorParams1D=off  ShowAdditionalParam=off  OutDataTypeStr=double
  accel_error1 : DataStoreMemory  DataStoreName=accel_error  ReadBeforeWriteMsg=warning  WriteAfterWriteMsg=warning  WriteAfterReadMsg=warning  InitialValue=accel_error  VectorParams1D=off  ShowAdditionalParam=off  OutDataTypeStr=double
  accel_last_z_cms1 : DataStoreMemory  DataStoreName=accel_last_z_cms  ReadBeforeWriteMsg=warning  WriteAfterWriteMsg=warning  WriteAfterReadMsg=warning  InitialValue=accel_last_z_cms  VectorParams1D=off  ShowAdditionalParam=off  OutDataTypeStr=double
  accel_pitch_max1 : DataStoreMemory  DataStoreName=accel_pitch_max  ReadBeforeWriteMsg=warning  WriteAfterWriteMsg=warning  WriteAfterReadMsg=warning  InitialValue=accel_pitch_max  VectorParams1D=off  ShowAdditionalParam=off  OutDataTypeStr=double
  accel_roll_max1 : DataStoreMemory  DataStoreName=accel_roll_max  ReadBeforeWriteMsg=warning  WriteAfterWriteMsg=warning  WriteAfterReadMsg=warning  InitialValue=accel_roll_max  VectorParams1D=off  ShowAdditionalParam=off  OutDataTypeStr=double
  accel_target1 : DataStoreMemory  DataStoreName=accel_target  ReadBeforeWriteMsg=warning  WriteAfterWriteMsg=warning  WriteAfterReadMsg=warning  InitialValue=accel_target  VectorParams1D=off  ShowAdditionalParam=off  OutDataTypeStr=double
  accel_x1 : DataStoreMemory  DataStoreName=accel_x  ReadBeforeWriteMsg=warning  WriteAfterWriteMsg=warning  WriteAfterReadMsg=warning  InitialValue=accel_x  ShowAdditionalParam=off  OutDataTypeStr=double
  accel_xy_angle_max1 : DataStoreMemory  DataStoreName=accel_xy_angle_max  ReadBeforeWriteMsg=warning  WriteAfterWriteMsg=warning  WriteAfterReadMsg=warning  InitialValue=accel_xy_angle_max  VectorParams1D=off  ShowAdditionalParam=off  OutDataTypeStr=double
  accel_xy_input1 : DataStoreMemory  DataStoreName=accel_xy_input  ReadBeforeWriteMsg=warning  WriteAfterWriteMsg=warning  WriteAfterReadMsg=warning  InitialValue=accel_xy_input  VectorParams1D=off  ShowAdditionalParam=off  OutDataTypeStr=double
  accel_y1 : DataStoreMemory  DataStoreName=accel_y  ReadBeforeWriteMsg=warning  WriteAfterWriteMsg=warning  WriteAfterReadMsg=warning  InitialValue=accel_y  ShowAdditionalParam=off  OutDataTypeStr=double
  accel_yaw_max1 : DataStoreMemory  DataStoreName=accel_yaw_max  ReadBeforeWriteMsg=warning  WriteAfterWriteMsg=warning  WriteAfterReadMsg=warning  InitialValue=accel_yaw_max  VectorParams1D=off  ShowAdditionalParam=off  OutDataTypeStr=double
  accel_z1 : DataStoreMemory  DataStoreName=accel_z  ReadBeforeWriteMsg=warning  WriteAfterWriteMsg=warning  WriteAfterReadMsg=warning  InitialValue=accel_z  ShowAdditionalParam=off  OutDataTypeStr=double
  aerodynamic_load_factor1 : DataStoreMemory  DataStoreName=aerodynamic_load_factor  ReadBeforeWriteMsg=warning  WriteAfterWriteMsg=warning  WriteAfterReadMsg=warning  InitialValue=aerodynamic_load_factor  ShowAdditionalParam=off  OutDataTypeStr=double
  air_density_ratio1 : DataStoreMemory  DataStoreName=air_density_ratio  ReadBeforeWriteMsg=warning  WriteAfterWriteMsg=warning  WriteAfterReadMsg=warning  InitialValue=air_density_ratio  VectorParams1D=off  ShowAdditionalParam=off  OutDataTypeStr=double
  airspeed_max1 : DataStoreMemory  DataStoreName=airspeed_max  ReadBeforeWriteMsg=warning  WriteAfterWriteMsg=warning  WriteAfterReadMsg=warning  InitialValue=airspeed_max  VectorParams1D=off  ShowAdditionalParam=off  OutDataTypeStr=double
  airspeed_min1 : DataStoreMemory  DataStoreName=airspeed_min  ReadBeforeWriteMsg=warning  WriteAfterWriteMsg=warning  WriteAfterReadMsg=warning  InitialValue=airspeed_min  VectorParams1D=off  ShowAdditionalParam=off  OutDataTypeStr=double
  althold_lean_angle_max1 : DataStoreMemory  DataStoreName=althold_lean_angle_max  ReadBeforeWriteMsg=warning  WriteAfterWriteMsg=warning  WriteAfterReadMsg=warning  InitialValue=althold_lean_angle_max  VectorParams1D=off  ShowAdditionalParam=off  OutDataTypeStr=double
  ang_vel_pitch_max1 : DataStoreMemory  DataStoreName=ang_vel_pitch_max  ReadBeforeWriteMsg=warning  WriteAfterWriteMsg=warning  WriteAfterReadMsg=warning  InitialValue=ang_vel_pitch_max  ShowAdditionalParam=off  OutDataTypeStr=double
  ang_vel_roll_max1 : DataStoreMemory  DataStoreName=ang_vel_roll_max  ReadBeforeWriteMsg=warning  WriteAfterWriteMsg=warning  WriteAfterReadMsg=warning  InitialValue=ang_vel_roll_max  ShowAdditionalParam=off  OutDataTypeStr=double
  ang_vel_yaw_max1 : DataStoreMemory  DataStoreName=ang_vel_yaw_max  ReadBeforeWriteMsg=warning  WriteAfterWriteMsg=warning  WriteAfterReadMsg=warning  InitialValue=ang_vel_yaw_max  ShowAdditionalParam=off  OutDataTypeStr=double
  angle_boost1 : DataStoreMemory  DataStoreName=angle_boost  ReadBeforeWriteMsg=warning  WriteAfterWriteMsg=warning  WriteAfterReadMsg=warning  InitialValue=angle_boost  VectorParams1D=off  ShowAdditionalParam=off  OutDataTypeStr=double
  angle_boost_enabled1 : DataStoreMemory  DataStoreName=angle_boost_enabled  ReadBeforeWriteMsg=warning  WriteAfterWriteMsg=warning  WriteAfterReadMsg=warning  InitialValue=angle_boost_enabled  VectorParams1D=off  ShowAdditionalParam=off  OutDataTypeStr=double
  angle_limit_tc1 : DataStoreMemory  DataStoreName=angle_limit_tc  ReadBeforeWriteMsg=warning  WriteAfterWriteMsg=warning  WriteAfterReadMsg=warning  InitialValue=angle_limit_tc  VectorParams1D=off  ShowAdditionalParam=off  OutDataTypeStr=double
  armed1 : DataStoreMemory  DataStoreName=armed  ReadBeforeWriteMsg=warning  WriteAfterWriteMsg=warning  WriteAfterReadMsg=warning  InitialValue=armed  VectorParams1D=off  ShowAdditionalParam=off  OutDataTypeStr=double
  arspeed_filt1 : DataStoreMemory  DataStoreName=arspeed_filt  ReadBeforeWriteMsg=warning  WriteAfterWriteMsg=warning  WriteAfterReadMsg=warning  InitialValue=arspeed_filt  VectorParams1D=off  ShowAdditionalParam=off  OutDataTypeStr=double
  arspeed_temp1 : DataStoreMemory  DataStoreName=arspeed_temp  ReadBeforeWriteMsg=warning  WriteAfterWriteMsg=warning  WriteAfterReadMsg=warning  InitialValue=arspeed_temp  VectorParams1D=off  ShowAdditionalParam=off  OutDataTypeStr=double
  aspeed1 : DataStoreMemory  DataStoreName=aspeed  ReadBeforeWriteMsg=warning  WriteAfterWriteMsg=warning  WriteAfterReadMsg=warning  InitialValue=aspeed  ShowAdditionalParam=off  OutDataTypeStr=double
  aspeed_c2p1 : DataStoreMemory  DataStoreName=aspeed_c2p  ReadBeforeWriteMsg=warning  WriteAfterWriteMsg=warning  WriteAfterReadMsg=warning  InitialValue=aspeed_c2p  VectorParams1D=off  ShowAdditionalParam=off  OutDataTypeStr=double
  aspeed_c2ps1 : DataStoreMemory  DataStoreName=aspeed_c2ps  ReadBeforeWriteMsg=warning  WriteAfterWriteMsg=warning  WriteAfterReadMsg=warning  InitialValue=aspeed_c2ps  VectorParams1D=off  ShowAdditionalParam=off  OutDataTypeStr=double
  aspeed_cp1 : DataStoreMemory  DataStoreName=aspeed_cp  ReadBeforeWriteMsg=warning  WriteAfterWriteMsg=warning  WriteAfterReadMsg=warning  InitialValue=aspeed_cp  VectorParams1D=off  ShowAdditionalParam=off  OutDataTypeStr=double
  attitude_ang_error1 : DataStoreMemory  DataStoreName=attitude_ang_error  ReadBeforeWriteMsg=warning  WriteAfterWriteMsg=warning  WriteAfterReadMsg=warning  InitialValue=attitude_ang_error  VectorParams1D=off  ShowAdditionalParam=off  OutDataTypeStr=double
  attitude_error_vector1 : DataStoreMemory  DataStoreName=attitude_error_vector  ReadBeforeWriteMsg=warning  WriteAfterWriteMsg=warning  WriteAfterReadMsg=warning  InitialValue=attitude_error_vector  VectorParams1D=off  ShowAdditionalParam=off  OutDataTypeStr=double
  attitude_target_ang_vel1 : DataStoreMemory  DataStoreName=attitude_target_ang_vel  ReadBeforeWriteMsg=warning  WriteAfterWriteMsg=warning  WriteAfterReadMsg=warning  InitialValue=attitude_target_ang_vel  VectorParams1D=off  ShowAdditionalParam=off  OutDataTypeStr=double
  attitude_target_euler_angle1 : DataStoreMemory  DataStoreName=attitude_target_euler_angle  ReadBeforeWriteMsg=warning  WriteAfterWriteMsg=warning  WriteAfterReadMsg=warning  InitialValue=attitude_target_euler_angle  VectorParams1D=off  ShowAdditionalParam=off  OutDataTypeStr=double
  attitude_target_euler_rate1 : DataStoreMemory  DataStoreName=attitude_target_euler_rate  ReadBeforeWriteMsg=warning  WriteAfterWriteMsg=warning  WriteAfterReadMsg=warning  InitialValue=attitude_target_euler_rate  VectorParams1D=off  ShowAdditionalParam=off  OutDataTypeStr=double
  attitude_target_quat1 : DataStoreMemory  DataStoreName=attitude_target_quat  ReadBeforeWriteMsg=warning  WriteAfterWriteMsg=warning  WriteAfterReadMsg=warning  InitialValue=attitude_target_quat  VectorParams1D=off  ShowAdditionalParam=off  OutDataTypeStr=double
  bearing_error1 : DataStoreMemory  DataStoreName=bearing_error  ReadBeforeWriteMsg=warning  WriteAfterWriteMsg=warning  WriteAfterReadMsg=warning  InitialValue=bearing_error  VectorParams1D=off  ShowAdditionalParam=off  OutDataTypeStr=double
  center_WP1 : DataStoreMemory  DataStoreName=center_WP  ReadBeforeWriteMsg=warning  WriteAfterWriteMsg=warning  WriteAfterReadMsg=warning  InitialValue=center_WP  VectorParams1D=off  ShowAdditionalParam=off  OutDataTypeStr=double
  climb_rate1 : DataStoreMemory  DataStoreName=climb_rate  ReadBeforeWriteMsg=warning  WriteAfterWriteMsg=warning  WriteAfterReadMsg=warning  InitialValue=climb_rate  VectorParams1D=off  ShowAdditionalParam=off  OutDataTypeStr=double
  climb_rate_cms1 : DataStoreMemory  DataStoreName=climb_rate_cms  ReadBeforeWriteMsg=warning  WriteAfterWriteMsg=warning  WriteAfterReadMsg=warning  InitialValue=climb_rate_cms  VectorParams1D=off  ShowAdditionalParam=off  OutDataTypeStr=double
  crosstrack_error1 : DataStoreMemory  DataStoreName=crosstrack_error  ReadBeforeWriteMsg=warning  WriteAfterWriteMsg=warning  WriteAfterReadMsg=warning  InitialValue=crosstrack_error  VectorParams1D=off  ShowAdditionalParam=off  OutDataTypeStr=double
  curr_alt1 : DataStoreMemory  DataStoreName=curr_alt  ReadBeforeWriteMsg=warning  WriteAfterWriteMsg=warning  WriteAfterReadMsg=warning  InitialValue=curr_alt  VectorParams1D=off  ShowAdditionalParam=off  OutDataTypeStr=double
  curr_pos1 : DataStoreMemory  DataStoreName=curr_pos  ReadBeforeWriteMsg=warning  WriteAfterWriteMsg=warning  WriteAfterReadMsg=warning  InitialValue=curr_pos  ShowAdditionalParam=off  OutDataTypeStr=double
  curr_vel1 : DataStoreMemory  DataStoreName=curr_vel  ReadBeforeWriteMsg=warning  WriteAfterWriteMsg=warning  WriteAfterReadMsg=warning  InitialValue=curr_vel  VectorParams1D=off  ShowAdditionalParam=off  OutDataTypeStr=double
  current_loc1 : DataStoreMemory  DataStoreName=current_loc  ReadBeforeWriteMsg=warning  WriteAfterWriteMsg=warning  WriteAfterReadMsg=warning  InitialValue=current_loc  VectorParams1D=off  ShowAdditionalParam=off  OutDataTypeStr=double
  current_tilt1 : DataStoreMemory  DataStoreName=current_tilt  ReadBeforeWriteMsg=warning  WriteAfterWriteMsg=warning  WriteAfterReadMsg=warning  InitialValue=current_tilt  VectorParams1D=off  ShowAdditionalParam=off  OutDataTypeStr=double
  data_is_stale1 : DataStoreMemory  DataStoreName=data_is_stale  ReadBeforeWriteMsg=warning  WriteAfterWriteMsg=warning  WriteAfterReadMsg=warning  InitialValue=data_is_stale  VectorParams1D=off  ShowAdditionalParam=off  OutDataTypeStr=double
  desired_rate_pitch1 : DataStoreMemory  DataStoreName=desired_rate_pitch  ReadBeforeWriteMsg=warning  WriteAfterWriteMsg=warning  WriteAfterReadMsg=warning  InitialValue=desired_rate_pitch  VectorParams1D=off  ShowAdditionalParam=off  OutDataTypeStr=double
  desired_rate_roll1 : DataStoreMemory  DataStoreName=desired_rate_roll  ReadBeforeWriteMsg=warning  WriteAfterWriteMsg=warning  WriteAfterReadMsg=warning  InitialValue=desired_rate_roll  VectorParams1D=off  ShowAdditionalParam=off  OutDataTypeStr=double
  disable_integrator_pitch1 : DataStoreMemory  DataStoreName=disable_integrator_pitch  ReadBeforeWriteMsg=warning  WriteAfterWriteMsg=warning  WriteAfterReadMsg=warning  InitialValue=disable_integrator_pitch  ShowAdditionalParam=off  OutDataTypeStr=double
  disable_integrator_roll1 : DataStoreMemory  DataStoreName=disable_integrator_roll  ReadBeforeWriteMsg=warning  WriteAfterWriteMsg=warning  WriteAfterReadMsg=warning  InitialValue=disable_integrator_roll  ShowAdditionalParam=off  OutDataTypeStr=double
  disable_integrator_yaw1 : DataStoreMemory  DataStoreName=disable_integrator_yaw  ReadBeforeWriteMsg=warning  WriteAfterWriteMsg=warning  WriteAfterReadMsg=warning  InitialValue=disable_integrator_yaw  ShowAdditionalParam=off  OutDataTypeStr=double
  dist_min1 : DataStoreMemory  DataStoreName=dist_min  ReadBeforeWriteMsg=warning  WriteAfterWriteMsg=warning  WriteAfterReadMsg=warning  InitialValue=dist_min  VectorParams1D=off  ShowAdditionalParam=off  OutDataTypeStr=double
  dt1 : DataStoreMemory  DataStoreName=dt  ReadBeforeWriteMsg=warning  WriteAfterWriteMsg=warning  WriteAfterReadMsg=warning  InitialValue=dt  ShowAdditionalParam=off  OutDataTypeStr=double
  ff_throttle : DataStoreMemory  DataStoreName=ff_throttle  ReadBeforeWriteMsg=warning  WriteAfterWriteMsg=warning  WriteAfterReadMsg=warning  InitialValue=ff_throttle  VectorParams1D=off  ShowAdditionalParam=off  OutDataTypeStr=double
  freeze_ff_z1 : DataStoreMemory  DataStoreName=freeze_ff_z  ReadBeforeWriteMsg=warning  WriteAfterWriteMsg=warning  WriteAfterReadMsg=warning  InitialValue=freeze_ff_z  VectorParams1D=off  ShowAdditionalParam=off  OutDataTypeStr=double
  gains_D_pitch1 : DataStoreMemory  DataStoreName=gains_D_pitch  ReadBeforeWriteMsg=warning  WriteAfterWriteMsg=warning  WriteAfterReadMsg=warning  InitialValue=gains_D_pitch  ShowAdditionalParam=off  OutDataTypeStr=double
  gains_D_roll1 : DataStoreMemory  DataStoreName=gains_D_roll  ReadBeforeWriteMsg=warning  WriteAfterWriteMsg=warning  WriteAfterReadMsg=warning  InitialValue=gains_D_roll  ShowAdditionalParam=off  OutDataTypeStr=double
  gains_FF1 : DataStoreMemory  DataStoreName=gains_FF_pitch  ReadBeforeWriteMsg=warning  WriteAfterWriteMsg=warning  WriteAfterReadMsg=warning  InitialValue=gains_FF_pitch  ShowAdditionalParam=off  OutDataTypeStr=double
  gains_FF_roll1 : DataStoreMemory  DataStoreName=gains_FF_roll  ReadBeforeWriteMsg=warning  WriteAfterWriteMsg=warning  WriteAfterReadMsg=warning  InitialValue=gains_FF_roll  ShowAdditionalParam=off  OutDataTypeStr=double
  gains_I_pitch1 : DataStoreMemory  DataStoreName=gains_I_pitch  ReadBeforeWriteMsg=warning  WriteAfterWriteMsg=warning  WriteAfterReadMsg=warning  InitialValue=gains_I_pitch  ShowAdditionalParam=off  OutDataTypeStr=double
  gains_I_roll1 : DataStoreMemory  DataStoreName=gains_I_roll  ReadBeforeWriteMsg=warning  WriteAfterWriteMsg=warning  WriteAfterReadMsg=warning  InitialValue=gains_I_roll  ShowAdditionalParam=off  OutDataTypeStr=double
  gains_P1 : DataStoreMemory  DataStoreName=gains_P_pitch  ReadBeforeWriteMsg=warning  WriteAfterWriteMsg=warning  WriteAfterReadMsg=warning  InitialValue=gains_P_pitch  ShowAdditionalParam=off  OutDataTypeStr=double
  gains_P_roll1 : DataStoreMemory  DataStoreName=gains_P_roll  ReadBeforeWriteMsg=warning  WriteAfterWriteMsg=warning  WriteAfterReadMsg=warning  InitialValue=gains_P_roll  ShowAdditionalParam=off  OutDataTypeStr=double
  gains_imax_pitch1 : DataStoreMemory  DataStoreName=gains_imax_pitch  ReadBeforeWriteMsg=warning  WriteAfterWriteMsg=warning  WriteAfterReadMsg=warning  InitialValue=gains_imax_pitch  ShowAdditionalParam=off  OutDataTypeStr=double
  gains_imax_roll1 : DataStoreMemory  DataStoreName=gains_imax_roll  ReadBeforeWriteMsg=warning  WriteAfterWriteMsg=warning  WriteAfterReadMsg=warning  InitialValue=gains_imax_roll  ShowAdditionalParam=off  OutDataTypeStr=double
  gains_rmax1 : DataStoreMemory  DataStoreName=gains_rmax_roll  ReadBeforeWriteMsg=warning  WriteAfterWriteMsg=warning  WriteAfterReadMsg=warning  InitialValue=gains_rmax_roll  ShowAdditionalParam=off  OutDataTypeStr=double
  gains_rmax_pitch1 : DataStoreMemory  DataStoreName=gains_rmax_pitch  ReadBeforeWriteMsg=warning  WriteAfterWriteMsg=warning  WriteAfterReadMsg=warning  InitialValue=gains_rmax_pitch  ShowAdditionalParam=off  OutDataTypeStr=double
  gains_tau_pitch1 : DataStoreMemory  DataStoreName=gains_tau_pitch  ReadBeforeWriteMsg=warning  WriteAfterWriteMsg=warning  WriteAfterReadMsg=warning  InitialValue=gains_tau_pitch  ShowAdditionalParam=off  OutDataTypeStr=double
  gains_tau_roll1 : DataStoreMemory  DataStoreName=gains_tau_roll  ReadBeforeWriteMsg=warning  WriteAfterWriteMsg=warning  WriteAfterReadMsg=warning  InitialValue=gains_tau_roll  ShowAdditionalParam=off  OutDataTypeStr=double
  groundspeed_vector1 : DataStoreMemory  DataStoreName=groundspeed_vector  ReadBeforeWriteMsg=warning  WriteAfterWriteMsg=warning  WriteAfterReadMsg=warning  InitialValue=groundspeed_vector  VectorParams1D=off  ShowAdditionalParam=off  OutDataTypeStr=double
  gyro_x1 : DataStoreMemory  DataStoreName=gyro_x  ReadBeforeWriteMsg=warning  WriteAfterWriteMsg=warning  WriteAfterReadMsg=warning  InitialValue=gyro_x  ShowAdditionalParam=off  OutDataTypeStr=double
  gyro_y1 : DataStoreMemory  DataStoreName=gyro_y  ReadBeforeWriteMsg=warning  WriteAfterWriteMsg=warning  WriteAfterReadMsg=warning  InitialValue=gyro_y  ShowAdditionalParam=off  OutDataTypeStr=double
  gyro_z1 : DataStoreMemory  DataStoreName=gyro_z  ReadBeforeWriteMsg=warning  WriteAfterWriteMsg=warning  WriteAfterReadMsg=warning  InitialValue=gyro_z  ShowAdditionalParam=off  OutDataTypeStr=double
  height1 : DataStoreMemory  DataStoreName=height  ReadBeforeWriteMsg=warning  WriteAfterWriteMsg=warning  WriteAfterReadMsg=warning  InitialValue=height  VectorParams1D=off  ShowAdditionalParam=off  OutDataTypeStr=double
  hgt_dem1 : DataStoreMemory  DataStoreName=hgt_dem  ReadBeforeWriteMsg=warning  WriteAfterWriteMsg=warning  WriteAfterReadMsg=warning  InitialValue=hgt_dem  VectorParams1D=off  ShowAdditionalParam=off  OutDataTypeStr=double
  hgt_dem_adj1 : DataStoreMemory  DataStoreName=hgt_dem_adj  ReadBeforeWriteMsg=warning  WriteAfterWriteMsg=warning  WriteAfterReadMsg=warning  InitialValue=hgt_dem_adj  VectorParams1D=off  ShowAdditionalParam=off  OutDataTypeStr=double
  hgt_dem_adj_last1 : DataStoreMemory  DataStoreName=hgt_dem_adj_last  ReadBeforeWriteMsg=warning  WriteAfterWriteMsg=warning  WriteAfterReadMsg=warning  InitialValue=hgt_dem_adj_last  VectorParams1D=off  ShowAdditionalParam=off  OutDataTypeStr=double
  hgt_dem_cm1 : DataStoreMemory  DataStoreName=hgt_dem_cm  ReadBeforeWriteMsg=warning  WriteAfterWriteMsg=warning  WriteAfterReadMsg=warning  InitialValue=hgt_dem_cm  VectorParams1D=off  ShowAdditionalParam=off  OutDataTypeStr=double
  hgt_dem_in_old1 : DataStoreMemory  DataStoreName=hgt_dem_in_old  ReadBeforeWriteMsg=warning  WriteAfterWriteMsg=warning  WriteAfterReadMsg=warning  InitialValue=hgt_dem_in_old  VectorParams1D=off  ShowAdditionalParam=off  OutDataTypeStr=double
  hgt_dem_prev1 : DataStoreMemory  DataStoreName=hgt_dem_prev  ReadBeforeWriteMsg=warning  WriteAfterWriteMsg=warning  WriteAfterReadMsg=warning  InitialValue=hgt_dem_prev  VectorParams1D=off  ShowAdditionalParam=off  OutDataTypeStr=double
  hgt_rate_dem1 : DataStoreMemory  DataStoreName=hgt_rate_dem  ReadBeforeWriteMsg=warning  WriteAfterWriteMsg=warning  WriteAfterReadMsg=warning  InitialValue=hgt_rate_dem  VectorParams1D=off  ShowAdditionalParam=off  OutDataTypeStr=double
  highest_airspeed1 : DataStoreMemory  DataStoreName=highest_airspeed  ReadBeforeWriteMsg=warning  WriteAfterWriteMsg=warning  WriteAfterReadMsg=warning  InitialValue=highest_airspeed  ShowAdditionalParam=off  OutDataTypeStr=double
  imax_yaw1 : DataStoreMemory  DataStoreName=imax_yaw  ReadBeforeWriteMsg=warning  WriteAfterWriteMsg=warning  WriteAfterReadMsg=warning  InitialValue=imax_yaw  ShowAdditionalParam=off  OutDataTypeStr=double
  inint1 : DataStoreMemory  DataStoreName=inint  ReadBeforeWriteMsg=warning  WriteAfterWriteMsg=warning  WriteAfterReadMsg=warning  InitialValue=inint  VectorParams1D=off  ShowAdditionalParam=off  OutDataTypeStr=double
  inint_hgt1 : DataStoreMemory  DataStoreName=inint_hgt  ReadBeforeWriteMsg=warning  WriteAfterWriteMsg=warning  WriteAfterReadMsg=warning  InitialValue=inint_hgt  VectorParams1D=off  ShowAdditionalParam=off  OutDataTypeStr=double
  input_euler_angle_roll_pitch_euler_rate_yaw4 : MATLAB Function  TreatAsAtomicUnit=on
  input_tc1 : DataStoreMemory  DataStoreName=input_tc  ReadBeforeWriteMsg=warning  WriteAfterWriteMsg=warning  WriteAfterReadMsg=warning  InitialValue=input_tc  VectorParams1D=off  ShowAdditionalParam=off  OutDataTypeStr=double
  integDTAS_state1 : DataStoreMemory  DataStoreName=integDTAS_state  ReadBeforeWriteMsg=warning  WriteAfterWriteMsg=warning  WriteAfterReadMsg=warning  InitialValue=integDTAS_state  VectorParams1D=off  ShowAdditionalParam=off  OutDataTypeStr=double
  integGain1 : DataStoreMemory  DataStoreName=integGain  ReadBeforeWriteMsg=warning  WriteAfterWriteMsg=warning  WriteAfterReadMsg=warning  InitialValue=integGain  VectorParams1D=off  ShowAdditionalParam=off  OutDataTypeStr=double
  integSEB_state1 : DataStoreMemory  DataStoreName=integSEB_state  ReadBeforeWriteMsg=warning  WriteAfterWriteMsg=warning  WriteAfterReadMsg=warning  InitialValue=integSEB_state  VectorParams1D=off  ShowAdditionalParam=off  OutDataTypeStr=double
  integTHR_state1 : DataStoreMemory  DataStoreName=integTHR_state  ReadBeforeWriteMsg=warning  WriteAfterWriteMsg=warning  WriteAfterReadMsg=warning  InitialValue=integTHR_state  VectorParams1D=off  ShowAdditionalParam=off  OutDataTypeStr=double
  integrator_yaw1 : DataStoreMemory  DataStoreName=integrator_yaw  ReadBeforeWriteMsg=warning  WriteAfterWriteMsg=warning  WriteAfterReadMsg=warning  InitialValue=integrator_yaw  ShowAdditionalParam=off  OutDataTypeStr=double
  inverted_flight1 : DataStoreMemory  DataStoreName=inverted_flight  ReadBeforeWriteMsg=warning  WriteAfterWriteMsg=warning  WriteAfterReadMsg=warning  InitialValue=inverted_flight  ShowAdditionalParam=off  OutDataTypeStr=double
  is_active_xy1 : DataStoreMemory  DataStoreName=is_active_xy  ReadBeforeWriteMsg=warning  WriteAfterWriteMsg=warning  WriteAfterReadMsg=warning  InitialValue=is_active_xy  VectorParams1D=off  ShowAdditionalParam=off  OutDataTypeStr=double
  is_active_z1 : DataStoreMemory  DataStoreName=is_active_z  ReadBeforeWriteMsg=warning  WriteAfterWriteMsg=warning  WriteAfterReadMsg=warning  InitialValue=is_active_z  VectorParams1D=off  ShowAdditionalParam=off  OutDataTypeStr=double
  k_aileron1 : DataStoreMemory  DataStoreName=k_aileron  ReadBeforeWriteMsg=warning  WriteAfterWriteMsg=warning  WriteAfterReadMsg=warning  InitialValue=k_aileron  ShowAdditionalParam=off  OutDataTypeStr=double
  k_elevator1 : DataStoreMemory  DataStoreName=k_elevator  ReadBeforeWriteMsg=warning  WriteAfterWriteMsg=warning  WriteAfterReadMsg=warning  InitialValue=k_elevator  ShowAdditionalParam=off  OutDataTypeStr=double
  k_rudder1 : DataStoreMemory  DataStoreName=k_rudder  ReadBeforeWriteMsg=warning  WriteAfterWriteMsg=warning  WriteAfterReadMsg=warning  InitialValue=k_rudder  ShowAdditionalParam=off  OutDataTypeStr=double
  k_throttle1 : DataStoreMemory  DataStoreName=k_throttle  ReadBeforeWriteMsg=warning  WriteAfterWriteMsg=warning  WriteAfterReadMsg=warning  InitialValue=k_throttle  ShowAdditionalParam=off  OutDataTypeStr=double
  k_throttle_c2p : DataStoreMemory  DataStoreName=k_throttle_c2p  ReadBeforeWriteMsg=warning  WriteAfterWriteMsg=warning  WriteAfterReadMsg=warning  InitialValue=k_throttle_c2p  VectorParams1D=off  ShowAdditionalParam=off  OutDataTypeStr=double
  kff_rudder_mix1 : DataStoreMemory  DataStoreName=kff_rudder_mix  ReadBeforeWriteMsg=warning  WriteAfterWriteMsg=warning  WriteAfterReadMsg=warning  InitialValue=kff_rudder_mix  ShowAdditionalParam=off  OutDataTypeStr=double
  kff_throttle_to_pitch1 : DataStoreMemory  DataStoreName=kff_throttle_to_pitch  ReadBeforeWriteMsg=warning  WriteAfterWriteMsg=warning  WriteAfterReadMsg=warning  InitialValue=kff_throttle_to_pitch  ShowAdditionalParam=off  OutDataTypeStr=double
  last_Nu1 : DataStoreMemory  DataStoreName=last_Nu  ReadBeforeWriteMsg=warning  WriteAfterWriteMsg=warning  WriteAfterReadMsg=warning  InitialValue=last_Nu  VectorParams1D=off  ShowAdditionalParam=off  OutDataTypeStr=double
  last_out_pitch1 : DataStoreMemory  DataStoreName=last_out_pitch  ReadBeforeWriteMsg=warning  WriteAfterWriteMsg=warning  WriteAfterReadMsg=warning  InitialValue=last_out_pitch  ShowAdditionalParam=off  OutDataTypeStr=double
  last_out_roll1 : DataStoreMemory  DataStoreName=last_out_roll  ReadBeforeWriteMsg=warning  WriteAfterWriteMsg=warning  WriteAfterReadMsg=warning  InitialValue=last_out_roll  ShowAdditionalParam=off  OutDataTypeStr=double
  last_out_yaw1 : DataStoreMemory  DataStoreName=last_out_yaw  ReadBeforeWriteMsg=warning  WriteAfterWriteMsg=warning  WriteAfterReadMsg=warning  InitialValue=last_out_yaw  ShowAdditionalParam=off  OutDataTypeStr=double
  last_pitch_dem1 : DataStoreMemory  DataStoreName=last_pitch_dem  ReadBeforeWriteMsg=warning  WriteAfterWriteMsg=warning  WriteAfterReadMsg=warning  InitialValue=last_pitch_dem  VectorParams1D=off  ShowAdditionalParam=off  OutDataTypeStr=double
  last_rate_hp_in_yaw1 : DataStoreMemory  DataStoreName=last_rate_hp_in_yaw  ReadBeforeWriteMsg=warning  WriteAfterWriteMsg=warning  WriteAfterReadMsg=warning  InitialValue=last_rate_hp_in_yaw  ShowAdditionalParam=off  OutDataTypeStr=double
  last_rate_hp_out_yaw1 : DataStoreMemory  DataStoreName=last_rate_hp_out_yaw  ReadBeforeWriteMsg=warning  WriteAfterWriteMsg=warning  WriteAfterReadMsg=warning  InitialValue=last_rate_hp_out_yaw  ShowAdditionalParam=off  OutDataTypeStr=double
  last_throttle_dem1 : DataStoreMemory  DataStoreName=last_throttle_dem  ReadBeforeWriteMsg=warning  WriteAfterWriteMsg=warning  WriteAfterReadMsg=warning  InitialValue=last_throttle_dem  VectorParams1D=off  ShowAdditionalParam=off  OutDataTypeStr=double
  latAccDem1 : DataStoreMemory  DataStoreName=latAccDem  ReadBeforeWriteMsg=warning  WriteAfterWriteMsg=warning  WriteAfterReadMsg=warning  InitialValue=latAccDem  VectorParams1D=off  ShowAdditionalParam=off  OutDataTypeStr=double
  leash1 : DataStoreMemory  DataStoreName=leash  ReadBeforeWriteMsg=warning  WriteAfterWriteMsg=warning  WriteAfterReadMsg=warning  InitialValue=POSCONTROL_LEASH_LENGTH_MIN  ShowAdditionalParam=off  OutDataTypeStr=double
  leash_down_z1 : DataStoreMemory  DataStoreName=leash_down_z  ReadBeforeWriteMsg=warning  WriteAfterWriteMsg=warning  WriteAfterReadMsg=warning  InitialValue=POSCONTROL_LEASH_LENGTH_MIN  ShowAdditionalParam=off  OutDataTypeStr=double
  leash_up_z1 : DataStoreMemory  DataStoreName=leash_up_z  ReadBeforeWriteMsg=warning  WriteAfterWriteMsg=warning  WriteAfterReadMsg=warning  InitialValue=POSCONTROL_LEASH_LENGTH_MIN  ShowAdditionalParam=off  OutDataTypeStr=double
  limit_accel_xy1 : DataStoreMemory  DataStoreName=limit_accel_xy  ReadBeforeWriteMsg=warning  WriteAfterWriteMsg=warning  WriteAfterReadMsg=warning  InitialValue=limit_accel_xy  VectorParams1D=off  ShowAdditionalParam=off  OutDataTypeStr=double
  limit_pos_down1 : DataStoreMemory  DataStoreName=limit_pos_down  ReadBeforeWriteMsg=warning  WriteAfterWriteMsg=warning  WriteAfterReadMsg=warning  InitialValue=limit_pos_down  VectorParams1D=off  ShowAdditionalParam=off  OutDataTypeStr=double
  limit_pos_up1 : DataStoreMemory  DataStoreName=limit_pos_up  ReadBeforeWriteMsg=warning  WriteAfterWriteMsg=warning  WriteAfterReadMsg=warning  InitialValue=limit_pos_up  VectorParams1D=off  ShowAdditionalParam=off  OutDataTypeStr=double
  limit_roll_pitch1 : DataStoreMemory  DataStoreName=limit_roll_pitch  ReadBeforeWriteMsg=warning  WriteAfterWriteMsg=warning  WriteAfterReadMsg=warning  InitialValue=limit_roll_pitch  VectorParams1D=off  ShowAdditionalParam=off  OutDataTypeStr=double
  limit_vel_down1 : DataStoreMemory  DataStoreName=limit_vel_down  ReadBeforeWriteMsg=warning  WriteAfterWriteMsg=warning  WriteAfterReadMsg=warning  InitialValue=limit_vel_down  VectorParams1D=off  ShowAdditionalParam=off  OutDataTypeStr=double
  limit_vel_up1 : DataStoreMemory  DataStoreName=limit_vel_up  ReadBeforeWriteMsg=warning  WriteAfterWriteMsg=warning  WriteAfterReadMsg=warning  InitialValue=limit_vel_up  ShowAdditionalParam=off  OutDataTypeStr=double
  limit_yaw1 : DataStoreMemory  DataStoreName=limit_yaw  ReadBeforeWriteMsg=warning  WriteAfterWriteMsg=warning  WriteAfterReadMsg=warning  InitialValue=limit_yaw  VectorParams1D=off  ShowAdditionalParam=off  OutDataTypeStr=double
  loc1 : DataStoreMemory  DataStoreName=loc  ReadBeforeWriteMsg=warning  WriteAfterWriteMsg=warning  WriteAfterReadMsg=warning  InitialValue=loc  VectorParams1D=off  ShowAdditionalParam=off  OutDataTypeStr=Bus: Bus_wp
  loc_origin1 : DataStoreMemory  DataStoreName=loc_origin  ReadBeforeWriteMsg=warning  WriteAfterWriteMsg=warning  WriteAfterReadMsg=warning  InitialValue=loc_origin  VectorParams1D=off  ShowAdditionalParam=off  OutDataTypeStr=double
  loiter_bank_limit1 : DataStoreMemory  DataStoreName=loiter_bank_limit  ReadBeforeWriteMsg=warning  WriteAfterWriteMsg=warning  WriteAfterReadMsg=warning  InitialValue=loiter_bank_limit  VectorParams1D=off  ShowAdditionalParam=off  OutDataTypeStr=double
  loiter_direction1 : DataStoreMemory  DataStoreName=loiter_direction  ReadBeforeWriteMsg=warning  WriteAfterWriteMsg=warning  WriteAfterReadMsg=warning  InitialValue=loiter_direction  VectorParams1D=off  ShowAdditionalParam=off  OutDataTypeStr=double
  maxClimbRate1 : DataStoreMemory  DataStoreName=maxClimbRate  ReadBeforeWriteMsg=warning  WriteAfterWriteMsg=warning  WriteAfterReadMsg=warning  InitialValue=maxClimbRate  VectorParams1D=off  ShowAdditionalParam=off  OutDataTypeStr=double
  maxSinkRate1 : DataStoreMemory  DataStoreName=maxSinkRate  ReadBeforeWriteMsg=warning  WriteAfterWriteMsg=warning  WriteAfterReadMsg=warning  InitialValue=maxSinkRate  VectorParams1D=off  ShowAdditionalParam=off  OutDataTypeStr=double
  max_rate_neg1 : DataStoreMemory  DataStoreName=max_rate_neg  ReadBeforeWriteMsg=warning  WriteAfterWriteMsg=warning  WriteAfterReadMsg=warning  InitialValue=max_rate_neg  ShowAdditionalParam=off  OutDataTypeStr=double
  minSinkRate1 : DataStoreMemory  DataStoreName=minSinkRate  ReadBeforeWriteMsg=warning  WriteAfterWriteMsg=warning  WriteAfterReadMsg=warning  InitialValue=minSinkRate  VectorParams1D=off  ShowAdditionalParam=off  OutDataTypeStr=double
  mode1 : DataStoreMemory  DataStoreName=mode  ReadBeforeWriteMsg=warning  WriteAfterWriteMsg=warning  WriteAfterReadMsg=warning  InitialValue=mode  VectorParams1D=off  ShowAdditionalParam=off  OutDataTypeStr=double
  mode_L2 : DataStoreMemory  DataStoreName=mode_L1  ReadBeforeWriteMsg=warning  WriteAfterWriteMsg=warning  WriteAfterReadMsg=warning  InitialValue=mode_L1  VectorParams1D=off  ShowAdditionalParam=off  OutDataTypeStr=double
  motors_limit_roll_pitch1 : DataStoreMemory  DataStoreName=motors_limit_roll_pitch  ReadBeforeWriteMsg=warning  WriteAfterWriteMsg=warning  WriteAfterReadMsg=warning  InitialValue=motors_limit_roll_pitch  VectorParams1D=off  ShowAdditionalParam=off  OutDataTypeStr=double
  motors_limit_throttle_upper1 : DataStoreMemory  DataStoreName=motors_limit_throttle_upper  ReadBeforeWriteMsg=warning  WriteAfterWriteMsg=warning  WriteAfterReadMsg=warning  InitialValue=motors_limit_throttle_upper  VectorParams1D=off  ShowAdditionalParam=off  OutDataTypeStr=double
  motors_limit_yaw1 : DataStoreMemory  DataStoreName=motors_limit_yaw  ReadBeforeWriteMsg=warning  WriteAfterWriteMsg=warning  WriteAfterReadMsg=warning  InitialValue=motors_limit_yaw  VectorParams1D=off  ShowAdditionalParam=off  OutDataTypeStr=double
  nav_bearing1 : DataStoreMemory  DataStoreName=nav_bearing  ReadBeforeWriteMsg=warning  WriteAfterWriteMsg=warning  WriteAfterReadMsg=warning  InitialValue=nav_bearing  VectorParams1D=off  ShowAdditionalParam=off  OutDataTypeStr=double
  nav_pitch_cd1 : DataStoreMemory  DataStoreName=nav_pitch_cd  ReadBeforeWriteMsg=warning  WriteAfterWriteMsg=warning  WriteAfterReadMsg=warning  InitialValue=nav_pitch_cd  ShowAdditionalParam=off  OutDataTypeStr=double
  nav_roll_cd1 : DataStoreMemory  DataStoreName=nav_roll_cd  ReadBeforeWriteMsg=warning  WriteAfterWriteMsg=warning  WriteAfterReadMsg=warning  InitialValue=nav_roll_cd  ShowAdditionalParam=off  OutDataTypeStr=double
  next_WP1 : DataStoreMemory  DataStoreName=next_WP  ReadBeforeWriteMsg=warning  WriteAfterWriteMsg=warning  WriteAfterReadMsg=warning  InitialValue=next_WP  VectorParams1D=off  ShowAdditionalParam=off  OutDataTypeStr=double
  p_angle_pitch1 : DataStoreMemory  DataStoreName=p_angle_pitch  ReadBeforeWriteMsg=warning  WriteAfterWriteMsg=warning  WriteAfterReadMsg=warning  InitialValue=p_angle_pitch  VectorParams1D=off  ShowAdditionalParam=off  OutDataTypeStr=double
  p_angle_roll1 : DataStoreMemory  DataStoreName=p_angle_roll  ReadBeforeWriteMsg=warning  WriteAfterWriteMsg=warning  WriteAfterReadMsg=warning  InitialValue=p_angle_roll  ShowAdditionalParam=off  OutDataTypeStr=double
  p_angle_yaw1 : DataStoreMemory  DataStoreName=p_angle_yaw  ReadBeforeWriteMsg=warning  WriteAfterWriteMsg=warning  WriteAfterReadMsg=warning  InitialValue=p_angle_yaw  ShowAdditionalParam=off  OutDataTypeStr=double
  p_ff_throttle1 : DataStoreMemory  DataStoreName=p_ff_throttle  ReadBeforeWriteMsg=warning  WriteAfterWriteMsg=warning  WriteAfterReadMsg=warning  InitialValue=p_ff_throttle  VectorParams1D=off  ShowAdditionalParam=off  OutDataTypeStr=double
  p_plane_c2p1 : DataStoreMemory  DataStoreName=p_plane_c2p  ReadBeforeWriteMsg=warning  WriteAfterWriteMsg=warning  WriteAfterReadMsg=warning  InitialValue=p_plane_c2p  VectorParams1D=off  ShowAdditionalParam=off  OutDataTypeStr=double
  p_plane_cp1 : DataStoreMemory  DataStoreName=p_plane_cp  ReadBeforeWriteMsg=warning  WriteAfterWriteMsg=warning  WriteAfterReadMsg=warning  InitialValue=p_plane_cp  VectorParams1D=off  ShowAdditionalParam=off  OutDataTypeStr=double
  p_tail_tilt1 : DataStoreMemory  DataStoreName=p_tail_tilt  ReadBeforeWriteMsg=warning  WriteAfterWriteMsg=warning  WriteAfterReadMsg=warning  InitialValue=p_tail_tilt  VectorParams1D=off  ShowAdditionalParam=off  OutDataTypeStr=double
  p_tilt_pitch_target1 : DataStoreMemory  DataStoreName=p_tilt_pitch_target  ReadBeforeWriteMsg=warning  WriteAfterWriteMsg=warning  WriteAfterReadMsg=warning  InitialValue=p_tilt_pitch_target  VectorParams1D=off  ShowAdditionalParam=off  OutDataTypeStr=double
  pid_accel_z_derivative1 : DataStoreMemory  DataStoreName=pid_accel_z_derivative  ReadBeforeWriteMsg=warning  WriteAfterWriteMsg=warning  WriteAfterReadMsg=warning  InitialValue=pid_accel_z_derivative  VectorParams1D=off  ShowAdditionalParam=off  OutDataTypeStr=double
  pid_accel_z_input1 : DataStoreMemory  DataStoreName=pid_accel_z_input  ReadBeforeWriteMsg=warning  WriteAfterWriteMsg=warning  WriteAfterReadMsg=warning  InitialValue=pid_accel_z_input  VectorParams1D=off  ShowAdditionalParam=off  OutDataTypeStr=double
  pid_accel_z_integrator1 : DataStoreMemory  DataStoreName=pid_accel_z_integrator  ReadBeforeWriteMsg=warning  WriteAfterWriteMsg=warning  WriteAfterReadMsg=warning  InitialValue=pid_accel_z_integrator  VectorParams1D=off  ShowAdditionalParam=off  OutDataTypeStr=double
  pid_accel_z_reset_filter1 : DataStoreMemory  DataStoreName=pid_accel_z_reset_filter  ReadBeforeWriteMsg=warning  WriteAfterWriteMsg=warning  WriteAfterReadMsg=warning  InitialValue=pid_accel_z_reset_filter  VectorParams1D=off  ShowAdditionalParam=off  OutDataTypeStr=double
  pid_info_D_pitch1 : DataStoreMemory  DataStoreName=pid_info_D_pitch  ReadBeforeWriteMsg=warning  WriteAfterWriteMsg=warning  WriteAfterReadMsg=warning  InitialValue=pid_info_D_pitch  ShowAdditionalParam=off  OutDataTypeStr=double
  pid_info_D_roll1 : DataStoreMemory  DataStoreName=pid_info_D_roll  ReadBeforeWriteMsg=warning  WriteAfterWriteMsg=warning  WriteAfterReadMsg=warning  InitialValue=pid_info_D_roll  ShowAdditionalParam=off  OutDataTypeStr=double
  pid_info_D_yaw1 : DataStoreMemory  DataStoreName=pid_info_D_yaw  ReadBeforeWriteMsg=warning  WriteAfterWriteMsg=warning  WriteAfterReadMsg=warning  InitialValue=pid_info_D_yaw  ShowAdditionalParam=off  OutDataTypeStr=double
  pid_info_FF1 : DataStoreMemory  DataStoreName=pid_info_FF_pitch  ReadBeforeWriteMsg=warning  WriteAfterWriteMsg=warning  WriteAfterReadMsg=warning  InitialValue=pid_info_FF_pitch  ShowAdditionalParam=off  OutDataTypeStr=double
  pid_info_FF_roll1 : DataStoreMemory  DataStoreName=pid_info_FF_roll  ReadBeforeWriteMsg=warning  WriteAfterWriteMsg=warning  WriteAfterReadMsg=warning  InitialValue=pid_info_FF_roll  ShowAdditionalParam=off  OutDataTypeStr=double
  pid_info_I_pitch1 : DataStoreMemory  DataStoreName=pid_info_I_pitch  ReadBeforeWriteMsg=warning  WriteAfterWriteMsg=warning  WriteAfterReadMsg=warning  InitialValue=pid_info_I_pitch  ShowAdditionalParam=off  OutDataTypeStr=double
  pid_info_I_roll1 : DataStoreMemory  DataStoreName=pid_info_I_roll  ReadBeforeWriteMsg=warning  WriteAfterWriteMsg=warning  WriteAfterReadMsg=warning  InitialValue=pid_info_I_roll  ShowAdditionalParam=off  OutDataTypeStr=double
  pid_info_I_yaw1 : DataStoreMemory  DataStoreName=pid_info_I_yaw  ReadBeforeWriteMsg=warning  WriteAfterWriteMsg=warning  WriteAfterReadMsg=warning  InitialValue=pid_info_I_yaw  ShowAdditionalParam=off  OutDataTypeStr=double
  pid_info_P_pitch1 : DataStoreMemory  DataStoreName=pid_info_P_pitch  ReadBeforeWriteMsg=warning  WriteAfterWriteMsg=warning  WriteAfterReadMsg=warning  InitialValue=pid_info_P_pitch  ShowAdditionalParam=off  OutDataTypeStr=double
  pid_info_P_roll1 : DataStoreMemory  DataStoreName=pid_info_P_roll  ReadBeforeWriteMsg=warning  WriteAfterWriteMsg=warning  WriteAfterReadMsg=warning  InitialValue=pid_info_P_roll  ShowAdditionalParam=off  OutDataTypeStr=double
  pid_info_actua_pitchl1 : DataStoreMemory  DataStoreName=pid_info_actual_pitch  ReadBeforeWriteMsg=warning  WriteAfterWriteMsg=warning  WriteAfterReadMsg=warning  InitialValue=pid_info_actual_pitch  ShowAdditionalParam=off  OutDataTypeStr=double
  pid_info_actual_roll1 : DataStoreMemory  DataStoreName=pid_info_actual_roll  ReadBeforeWriteMsg=warning  WriteAfterWriteMsg=warning  WriteAfterReadMsg=warning  InitialValue=pid_info_actual_roll  ShowAdditionalParam=off  OutDataTypeStr=double
  pid_info_desired_pitch1 : DataStoreMemory  DataStoreName=pid_info_desired_pitch  ReadBeforeWriteMsg=warning  WriteAfterWriteMsg=warning  WriteAfterReadMsg=warning  InitialValue=pid_info_desired_pitch  ShowAdditionalParam=off  OutDataTypeStr=double
  pid_info_desired_roll1 : DataStoreMemory  DataStoreName=pid_info_desired_roll  ReadBeforeWriteMsg=warning  WriteAfterWriteMsg=warning  WriteAfterReadMsg=warning  InitialValue=pid_info_desired_roll  ShowAdditionalParam=off  OutDataTypeStr=double
  pid_vel_xy_derivative1 : DataStoreMemory  DataStoreName=pid_vel_xy_derivative  ReadBeforeWriteMsg=warning  WriteAfterWriteMsg=warning  WriteAfterReadMsg=warning  InitialValue=pid_vel_xy_derivative  VectorParams1D=off  ShowAdditionalParam=off  OutDataTypeStr=double
  pid_vel_xy_input1 : DataStoreMemory  DataStoreName=pid_vel_xy_input  ReadBeforeWriteMsg=warning  WriteAfterWriteMsg=warning  WriteAfterReadMsg=warning  InitialValue=pid_vel_xy_input  VectorParams1D=off  ShowAdditionalParam=off  OutDataTypeStr=double
  pid_vel_xy_integrator1 : DataStoreMemory  DataStoreName=pid_vel_xy_integrator  ReadBeforeWriteMsg=warning  WriteAfterWriteMsg=warning  WriteAfterReadMsg=warning  InitialValue=pid_vel_xy_integrator  VectorParams1D=off  ShowAdditionalParam=off  OutDataTypeStr=double
  pid_vel_xy_reset_filter1 : DataStoreMemory  DataStoreName=pid_vel_xy_reset_filter  ReadBeforeWriteMsg=warning  WriteAfterWriteMsg=warning  WriteAfterReadMsg=warning  InitialValue=pid_vel_xy_reset_filter  VectorParams1D=off  ShowAdditionalParam=off  OutDataTypeStr=double
  pitch1 : DataStoreMemory  DataStoreName=pitch  ReadBeforeWriteMsg=warning  WriteAfterWriteMsg=warning  WriteAfterReadMsg=warning  InitialValue=pitch  ShowAdditionalParam=off  OutDataTypeStr=double
  pitch_dem1 : DataStoreMemory  DataStoreName=pitch_dem  ReadBeforeWriteMsg=warning  WriteAfterWriteMsg=warning  WriteAfterReadMsg=warning  InitialValue=pitch_dem  VectorParams1D=off  ShowAdditionalParam=off  OutDataTypeStr=double
  pitch_dem_unc1 : DataStoreMemory  DataStoreName=pitch_dem_unc  ReadBeforeWriteMsg=warning  WriteAfterWriteMsg=warning  WriteAfterReadMsg=warning  InitialValue=pitch_dem_unc  VectorParams1D=off  ShowAdditionalParam=off  OutDataTypeStr=double
  pitch_factor1 : DataStoreMemory  DataStoreName=pitch_factor  ReadBeforeWriteMsg=warning  WriteAfterWriteMsg=warning  WriteAfterReadMsg=warning  InitialValue=pitch_factor  VectorParams1D=off  ShowAdditionalParam=off  OutDataTypeStr=double
  pitch_in1 : DataStoreMemory  DataStoreName=pitch_in  ReadBeforeWriteMsg=warning  WriteAfterWriteMsg=warning  WriteAfterReadMsg=warning  InitialValue=pitch_in  VectorParams1D=off  ShowAdditionalParam=off  OutDataTypeStr=double
  pitch_limit_max_cd1 : DataStoreMemory  DataStoreName=pitch_limit_max_cd  ReadBeforeWriteMsg=warning  WriteAfterWriteMsg=warning  WriteAfterReadMsg=warning  InitialValue=pitch_limit_max_cd  VectorParams1D=off  ShowAdditionalParam=off  OutDataTypeStr=double
  pitch_limit_min_cd1 : DataStoreMemory  DataStoreName=pitch_limit_min_cd  ReadBeforeWriteMsg=warning  WriteAfterWriteMsg=warning  WriteAfterReadMsg=warning  InitialValue=pitch_limit_min_cd  VectorParams1D=off  ShowAdditionalParam=off  OutDataTypeStr=double
  pitch_max1 : DataStoreMemory  DataStoreName=pitch_max  ReadBeforeWriteMsg=warning  WriteAfterWriteMsg=warning  WriteAfterReadMsg=warning  InitialValue=pitch_max  VectorParams1D=off  ShowAdditionalParam=off  OutDataTypeStr=double
  pitch_max_limit1 : DataStoreMemory  DataStoreName=pitch_max_limit  ReadBeforeWriteMsg=warning  WriteAfterWriteMsg=warning  WriteAfterReadMsg=warning  InitialValue=pitch_max_limit  VectorParams1D=off  ShowAdditionalParam=off  OutDataTypeStr=double
  pitch_min1 : DataStoreMemory  DataStoreName=pitch_min  ReadBeforeWriteMsg=warning  WriteAfterWriteMsg=warning  WriteAfterReadMsg=warning  InitialValue=pitch_min  VectorParams1D=off  ShowAdditionalParam=off  OutDataTypeStr=double
  pitch_target1 : DataStoreMemory  DataStoreName=pitch_target  ReadBeforeWriteMsg=warning  WriteAfterWriteMsg=warning  WriteAfterReadMsg=warning  InitialValue=pitch_target  VectorParams1D=off  ShowAdditionalParam=off  OutDataTypeStr=double
  pitch_target_c2p : DataStoreMemory  DataStoreName=pitch_target_c2p  ReadBeforeWriteMsg=warning  WriteAfterWriteMsg=warning  WriteAfterReadMsg=warning  InitialValue=pitch_target_c2p  VectorParams1D=off  ShowAdditionalParam=off  OutDataTypeStr=double
  pitch_target_p2c : DataStoreMemory  DataStoreName=pitch_target_p2c  ReadBeforeWriteMsg=warning  WriteAfterWriteMsg=warning  WriteAfterReadMsg=warning  InitialValue=pitch_target_p2c  VectorParams1D=off  ShowAdditionalParam=off  OutDataTypeStr=double
  pitch_target_pilot1 : DataStoreMemory  DataStoreName=pitch_target_pilot  ReadBeforeWriteMsg=warning  WriteAfterWriteMsg=warning  WriteAfterReadMsg=warning  InitialValue=pitch_target_pilot  VectorParams1D=off  ShowAdditionalParam=off  OutDataTypeStr=double
  plane_mode : DataStoreMemory  DataStoreName=plane_mode  ReadBeforeWriteMsg=warning  WriteAfterWriteMsg=warning  WriteAfterReadMsg=warning  InitialValue=plane_mode  VectorParams1D=off  ShowAdditionalParam=off  OutDataTypeStr=Enum: ENUM_plane_mode
  pos_error1 : DataStoreMemory  DataStoreName=pos_error  ReadBeforeWriteMsg=warning  WriteAfterWriteMsg=warning  WriteAfterReadMsg=warning  InitialValue=pos_error  VectorParams1D=off  ShowAdditionalParam=off  OutDataTypeStr=double
  pos_target1 : DataStoreMemory  DataStoreName=pos_target  ReadBeforeWriteMsg=warning  WriteAfterWriteMsg=warning  WriteAfterReadMsg=warning  InitialValue=pos_target  VectorParams1D=off  ShowAdditionalParam=off  OutDataTypeStr=double
  prev_WP1 : DataStoreMemory  DataStoreName=prev_WP  ReadBeforeWriteMsg=warning  WriteAfterWriteMsg=warning  WriteAfterReadMsg=warning  InitialValue=prev_WP  VectorParams1D=off  ShowAdditionalParam=off  OutDataTypeStr=double
  ptchDamp1 : DataStoreMemory  DataStoreName=ptchDamp  ReadBeforeWriteMsg=warning  WriteAfterWriteMsg=warning  WriteAfterReadMsg=warning  InitialValue=ptchDamp  VectorParams1D=off  ShowAdditionalParam=off  OutDataTypeStr=double
  pwm_max1 : DataStoreMemory  DataStoreName=pwm_max  ReadBeforeWriteMsg=warning  WriteAfterWriteMsg=warning  WriteAfterReadMsg=warning  InitialValue=pwm_max  ShowAdditionalParam=off  OutDataTypeStr=double
  pwm_min1 : DataStoreMemory  DataStoreName=pwm_min  ReadBeforeWriteMsg=warning  WriteAfterWriteMsg=warning  WriteAfterReadMsg=warning  InitialValue=pwm_min  ShowAdditionalParam=off  OutDataTypeStr=double
  pwm_out1 : DataStoreMemory  DataStoreName=pwm_out  ReadBeforeWriteMsg=warning  WriteAfterWriteMsg=warning  WriteAfterReadMsg=warning  InitialValue=pwm_out  ShowAdditionalParam=off  OutDataTypeStr=double
  pwm_tail : DataStoreMemory  DataStoreName=pwm_tail  ReadBeforeWriteMsg=warning  WriteAfterWriteMsg=warning  WriteAfterReadMsg=warning  InitialValue=pwm_tail  VectorParams1D=off  ShowAdditionalParam=off  OutDataTypeStr=double
  radius1 : DataStoreMemory  DataStoreName=radius  ReadBeforeWriteMsg=warning  WriteAfterWriteMsg=warning  WriteAfterReadMsg=warning  InitialValue=radius  VectorParams1D=off  ShowAdditionalParam=off  OutDataTypeStr=double
  rate_bf_ff_enabled1 : DataStoreMemory  DataStoreName=rate_bf_ff_enabled  ReadBeforeWriteMsg=warning  WriteAfterWriteMsg=warning  WriteAfterReadMsg=warning  InitialValue=rate_bf_ff_enabled  ShowAdditionalParam=off  OutDataTypeStr=double
  rate_pitch_pid_derivative1 : DataStoreMemory  DataStoreName=rate_pitch_pid_derivative  ReadBeforeWriteMsg=warning  WriteAfterWriteMsg=warning  WriteAfterReadMsg=warning  InitialValue=rate_pitch_pid_derivative  VectorParams1D=off  ShowAdditionalParam=off  OutDataTypeStr=double
  rate_pitch_pid_input1 : DataStoreMemory  DataStoreName=rate_pitch_pid_input  ReadBeforeWriteMsg=warning  WriteAfterWriteMsg=warning  WriteAfterReadMsg=warning  InitialValue=rate_pitch_pid_input  VectorParams1D=off  ShowAdditionalParam=off  OutDataTypeStr=double
  rate_pitch_pid_integrator1 : DataStoreMemory  DataStoreName=rate_pitch_pid_integrator  ReadBeforeWriteMsg=warning  WriteAfterWriteMsg=warning  WriteAfterReadMsg=warning  InitialValue=rate_pitch_pid_integrator  VectorParams1D=off  ShowAdditionalParam=off  OutDataTypeStr=double
  rate_pitch_pid_reset_filter1 : DataStoreMemory  DataStoreName=rate_pitch_pid_reset_filter  ReadBeforeWriteMsg=warning  WriteAfterWriteMsg=warning  WriteAfterReadMsg=warning  InitialValue=rate_pitch_pid_reset_filter  VectorParams1D=off  ShowAdditionalParam=off  OutDataTypeStr=double
  rate_roll_pid_derivative1 : DataStoreMemory  DataStoreName=rate_roll_pid_derivative  ReadBeforeWriteMsg=warning  WriteAfterWriteMsg=warning  WriteAfterReadMsg=warning  InitialValue=rate_roll_pid_derivative  VectorParams1D=off  ShowAdditionalParam=off  OutDataTypeStr=double
  rate_roll_pid_input1 : DataStoreMemory  DataStoreName=rate_roll_pid_input  ReadBeforeWriteMsg=warning  WriteAfterWriteMsg=warning  WriteAfterReadMsg=warning  InitialValue=rate_roll_pid_input  VectorParams1D=off  ShowAdditionalParam=off  OutDataTypeStr=double
  rate_roll_pid_integrator1 : DataStoreMemory  DataStoreName=rate_roll_pid_integrator  ReadBeforeWriteMsg=warning  WriteAfterWriteMsg=warning  WriteAfterReadMsg=warning  InitialValue=rate_roll_pid_integrator  VectorParams1D=off  ShowAdditionalParam=off  OutDataTypeStr=double
  rate_roll_pid_reset_filter1 : DataStoreMemory  DataStoreName=rate_roll_pid_reset_filter  ReadBeforeWriteMsg=warning  WriteAfterWriteMsg=warning  WriteAfterReadMsg=warning  InitialValue=rate_roll_pid_reset_filter  VectorParams1D=off  ShowAdditionalParam=off  OutDataTypeStr=double
  rate_target_ang_vel1 : DataStoreMemory  DataStoreName=rate_target_ang_vel  ReadBeforeWriteMsg=warning  WriteAfterWriteMsg=warning  WriteAfterReadMsg=warning  InitialValue=rate_target_ang_vel  VectorParams1D=off  ShowAdditionalParam=off  OutDataTypeStr=double
  rate_yaw_pid_derivative1 : DataStoreMemory  DataStoreName=rate_yaw_pid_derivative  ReadBeforeWriteMsg=warning  WriteAfterWriteMsg=warning  WriteAfterReadMsg=warning  InitialValue=rate_yaw_pid_derivative  VectorParams1D=off  ShowAdditionalParam=off  OutDataTypeStr=double
  rate_yaw_pid_input1 : DataStoreMemory  DataStoreName=rate_yaw_pid_input  ReadBeforeWriteMsg=warning  WriteAfterWriteMsg=warning  WriteAfterReadMsg=warning  InitialValue=rate_yaw_pid_input  VectorParams1D=off  ShowAdditionalParam=off  OutDataTypeStr=double
  rate_yaw_pid_integrator1 : DataStoreMemory  DataStoreName=rate_yaw_pid_integrator  ReadBeforeWriteMsg=warning  WriteAfterWriteMsg=warning  WriteAfterReadMsg=warning  InitialValue=rate_roll_pid_integrator  VectorParams1D=off  ShowAdditionalParam=off  OutDataTypeStr=double
  rate_yaw_pid_reset_filter1 : DataStoreMemory  DataStoreName=rate_yaw_pid_reset_filter  ReadBeforeWriteMsg=warning  WriteAfterWriteMsg=warning  WriteAfterReadMsg=warning  InitialValue=rate_yaw_pid_reset_filter  VectorParams1D=off  ShowAdditionalParam=off  OutDataTypeStr=double
  recalc_leash_xy1 : DataStoreMemory  DataStoreName=recalc_leash_xy  ReadBeforeWriteMsg=warning  WriteAfterWriteMsg=warning  WriteAfterReadMsg=warning  InitialValue=recalc_leash_xy  VectorParams1D=off  ShowAdditionalParam=off  OutDataTypeStr=double
  recalc_leash_z1 : DataStoreMemory  DataStoreName=recalc_leash_z  ReadBeforeWriteMsg=warning  WriteAfterWriteMsg=warning  WriteAfterReadMsg=warning  InitialValue=recalc_leash_z  ShowAdditionalParam=off  OutDataTypeStr=double
  reset_accel_to_lean_xy1 : DataStoreMemory  DataStoreName=reset_accel_to_lean_xy  ReadBeforeWriteMsg=warning  WriteAfterWriteMsg=warning  WriteAfterReadMsg=warning  InitialValue=reset_accel_to_lean_xy  VectorParams1D=off  ShowAdditionalParam=off  OutDataTypeStr=double
  reset_accel_to_throttle1 : DataStoreMemory  DataStoreName=reset_accel_to_throttle  ReadBeforeWriteMsg=warning  WriteAfterWriteMsg=warning  WriteAfterReadMsg=warning  InitialValue=reset_accel_to_throttle  VectorParams1D=off  ShowAdditionalParam=off  OutDataTypeStr=double
  reset_desired_vel_to_pos1 : DataStoreMemory  DataStoreName=reset_desired_vel_to_pos  ReadBeforeWriteMsg=warning  WriteAfterWriteMsg=warning  WriteAfterReadMsg=warning  InitialValue=reset_desired_vel_to_pos  VectorParams1D=off  ShowAdditionalParam=off  OutDataTypeStr=double
  reset_rate_to_accel_z1 : DataStoreMemory  DataStoreName=reset_rate_to_accel_z  ReadBeforeWriteMsg=warning  WriteAfterWriteMsg=warning  WriteAfterReadMsg=warning  InitialValue=reset_rate_to_accel_z  VectorParams1D=off  ShowAdditionalParam=off  OutDataTypeStr=double
  reverse1 : DataStoreMemory  DataStoreName=reverse  ReadBeforeWriteMsg=warning  WriteAfterWriteMsg=warning  WriteAfterReadMsg=warning  InitialValue=reverse  VectorParams1D=off  ShowAdditionalParam=off  OutDataTypeStr=double
  roll1 : DataStoreMemory  DataStoreName=roll  ReadBeforeWriteMsg=warning  WriteAfterWriteMsg=warning  WriteAfterReadMsg=warning  InitialValue=roll  ShowAdditionalParam=off  OutDataTypeStr=double
  rollComp1 : DataStoreMemory  DataStoreName=rollComp  ReadBeforeWriteMsg=warning  WriteAfterWriteMsg=warning  WriteAfterReadMsg=warning  InitialValue=rollComp  VectorParams1D=off  ShowAdditionalParam=off  OutDataTypeStr=double
  roll_factor1 : DataStoreMemory  DataStoreName=roll_factor  ReadBeforeWriteMsg=warning  WriteAfterWriteMsg=warning  WriteAfterReadMsg=warning  InitialValue=roll_factor  VectorParams1D=off  ShowAdditionalParam=off  OutDataTypeStr=double
  roll_ff_pitch1 : DataStoreMemory  DataStoreName=roll_ff_pitch  ReadBeforeWriteMsg=warning  WriteAfterWriteMsg=warning  WriteAfterReadMsg=warning  InitialValue=roll_ff_pitch  ShowAdditionalParam=off  OutDataTypeStr=double
  roll_ff_pitch_inint1 : DataStoreMemory  DataStoreName=roll_ff_pitch_inint  ReadBeforeWriteMsg=warning  WriteAfterWriteMsg=warning  WriteAfterReadMsg=warning  InitialValue=roll_ff_pitch_inint  VectorParams1D=off  ShowAdditionalParam=off  OutDataTypeStr=double
  roll_in1 : DataStoreMemory  DataStoreName=roll_in  ReadBeforeWriteMsg=warning  WriteAfterWriteMsg=warning  WriteAfterReadMsg=warning  InitialValue=roll_in  VectorParams1D=off  ShowAdditionalParam=off  OutDataTypeStr=double
  roll_limit_cd1 : DataStoreMemory  DataStoreName=roll_limit_cd  ReadBeforeWriteMsg=warning  WriteAfterWriteMsg=warning  WriteAfterReadMsg=warning  InitialValue=roll_limit_cd  ShowAdditionalParam=off  OutDataTypeStr=double
  roll_limit_cd_inint1 : DataStoreMemory  DataStoreName=roll_limit_cd_inint  ReadBeforeWriteMsg=warning  WriteAfterWriteMsg=warning  WriteAfterReadMsg=warning  InitialValue=roll_limit_cd_inint  ShowAdditionalParam=off  OutDataTypeStr=double
  roll_target1 : DataStoreMemory  DataStoreName=roll_target  ReadBeforeWriteMsg=warning  WriteAfterWriteMsg=warning  WriteAfterReadMsg=warning  InitialValue=roll_target  VectorParams1D=off  ShowAdditionalParam=off  OutDataTypeStr=double
  roll_target_pilot1 : DataStoreMemory  DataStoreName=roll_target_pilot  ReadBeforeWriteMsg=warning  WriteAfterWriteMsg=warning  WriteAfterReadMsg=warning  InitialValue=roll_target_pilot  VectorParams1D=off  ShowAdditionalParam=off  OutDataTypeStr=double
  rot_body_to_ned1 : DataStoreMemory  DataStoreName=rot_body_to_ned  ReadBeforeWriteMsg=warning  WriteAfterWriteMsg=warning  WriteAfterReadMsg=warning  InitialValue=rot_body_to_ned  VectorParams1D=off  ShowAdditionalParam=off  OutDataTypeStr=double
  scaling_speed1 : DataStoreMemory  DataStoreName=scaling_speed  ReadBeforeWriteMsg=warning  WriteAfterWriteMsg=warning  WriteAfterReadMsg=warning  InitialValue=scaling_speed  ShowAdditionalParam=off  OutDataTypeStr=double
  slew_yaw1 : DataStoreMemory  DataStoreName=slew_yaw  ReadBeforeWriteMsg=warning  WriteAfterWriteMsg=warning  WriteAfterReadMsg=warning  InitialValue=slew_yaw  VectorParams1D=off  ShowAdditionalParam=off  OutDataTypeStr=double
  smoothed_airspeed1 : DataStoreMemory  DataStoreName=smoothed_airspeed  ReadBeforeWriteMsg=warning  WriteAfterWriteMsg=warning  WriteAfterReadMsg=warning  InitialValue=smoothed_airspeed  ShowAdditionalParam=off  OutDataTypeStr=double
  spdCompFiltOmega1 : DataStoreMemory  DataStoreName=spdCompFiltOmega  ReadBeforeWriteMsg=warning  WriteAfterWriteMsg=warning  WriteAfterReadMsg=warning  InitialValue=spdCompFiltOmega  VectorParams1D=off  ShowAdditionalParam=off  OutDataTypeStr=double
  spdWeight1 : DataStoreMemory  DataStoreName=spdWeight  ReadBeforeWriteMsg=warning  WriteAfterWriteMsg=warning  WriteAfterReadMsg=warning  InitialValue=spdWeight  VectorParams1D=off  ShowAdditionalParam=off  OutDataTypeStr=double
  tail_tilt1 : DataStoreMemory  DataStoreName=tail_tilt  ReadBeforeWriteMsg=warning  WriteAfterWriteMsg=warning  WriteAfterReadMsg=warning  InitialValue=tail_tilt  VectorParams1D=off  ShowAdditionalParam=off  OutDataTypeStr=double
  tail_tilt_c2p1 : DataStoreMemory  DataStoreName=tail_tilt_c2p  ReadBeforeWriteMsg=warning  WriteAfterWriteMsg=warning  WriteAfterReadMsg=warning  InitialValue=tail_tilt_c2p  VectorParams1D=off  ShowAdditionalParam=off  OutDataTypeStr=double
  tail_tilt_p2c1 : DataStoreMemory  DataStoreName=tail_tilt_p2c  ReadBeforeWriteMsg=warning  WriteAfterWriteMsg=warning  WriteAfterReadMsg=warning  InitialValue=tail_tilt_p2c  VectorParams1D=off  ShowAdditionalParam=off  OutDataTypeStr=double
  tail_tilt_rate1 : DataStoreMemory  DataStoreName=tail_tilt_rate  ReadBeforeWriteMsg=warning  WriteAfterWriteMsg=warning  WriteAfterReadMsg=warning  InitialValue=tail_tilt_rate  VectorParams1D=off  ShowAdditionalParam=off  OutDataTypeStr=double
  take_off_land : DataStoreMemory  DataStoreName=take_off_land  ReadBeforeWriteMsg=warning  WriteAfterWriteMsg=warning  WriteAfterReadMsg=warning  InitialValue=take_off_land  VectorParams1D=off  ShowAdditionalParam=off  OutDataTypeStr=double
  target_bearing_cd1 : DataStoreMemory  DataStoreName=target_bearing_cd  ReadBeforeWriteMsg=warning  WriteAfterWriteMsg=warning  WriteAfterReadMsg=warning  InitialValue=target_bearing_cd  VectorParams1D=off  ShowAdditionalParam=off  OutDataTypeStr=double
  target_yaw_rate1 : DataStoreMemory  DataStoreName=target_yaw_rate  ReadBeforeWriteMsg=warning  WriteAfterWriteMsg=warning  WriteAfterReadMsg=warning  InitialValue=target_yaw_rate  VectorParams1D=off  ShowAdditionalParam=off  OutDataTypeStr=double
  thrDamp1 : DataStoreMemory  DataStoreName=thrDamp  ReadBeforeWriteMsg=warning  WriteAfterWriteMsg=warning  WriteAfterReadMsg=warning  InitialValue=thrDamp  VectorParams1D=off  ShowAdditionalParam=off  OutDataTypeStr=double
  thr_out_min : DataStoreMemory  DataStoreName=thr_out_min  ReadBeforeWriteMsg=warning  WriteAfterWriteMsg=warning  WriteAfterReadMsg=warning  InitialValue=thr_out_min  VectorParams1D=off  ShowAdditionalParam=off  OutDataTypeStr=double
  throttle_avg_max1 : DataStoreMemory  DataStoreName=throttle_avg_max  ReadBeforeWriteMsg=warning  WriteAfterWriteMsg=warning  WriteAfterReadMsg=warning  InitialValue=throttle_avg_max  VectorParams1D=off  ShowAdditionalParam=off  OutDataTypeStr=double
  throttle_cruise1 : DataStoreMemory  DataStoreName=throttle_cruise  ReadBeforeWriteMsg=warning  WriteAfterWriteMsg=warning  WriteAfterReadMsg=warning  InitialValue=throttle_cruise  VectorParams1D=off  ShowAdditionalParam=off  OutDataTypeStr=double
  throttle_cutoff_frequency1 : DataStoreMemory  DataStoreName=throttle_cutoff_frequency  ReadBeforeWriteMsg=warning  WriteAfterWriteMsg=warning  WriteAfterReadMsg=warning  InitialValue=throttle_cutoff_frequency  VectorParams1D=off  ShowAdditionalParam=off  OutDataTypeStr=double
  throttle_dem1 : DataStoreMemory  DataStoreName=throttle_dem  ReadBeforeWriteMsg=warning  WriteAfterWriteMsg=warning  WriteAfterReadMsg=warning  InitialValue=throttle_dem  VectorParams1D=off  ShowAdditionalParam=off  OutDataTypeStr=double
  throttle_filter1 : DataStoreMemory  DataStoreName=throttle_filter  ReadBeforeWriteMsg=warning  WriteAfterWriteMsg=warning  WriteAfterReadMsg=warning  InitialValue=throttle_filter  VectorParams1D=off  ShowAdditionalParam=off  OutDataTypeStr=double
  throttle_ground : DataStoreMemory  DataStoreName=throttle_ground  ReadBeforeWriteMsg=warning  WriteAfterWriteMsg=warning  WriteAfterReadMsg=warning  InitialValue=throttle_ground  VectorParams1D=off  ShowAdditionalParam=off  OutDataTypeStr=double
  throttle_hover1 : DataStoreMemory  DataStoreName=throttle_hover  ReadBeforeWriteMsg=warning  WriteAfterWriteMsg=warning  WriteAfterReadMsg=warning  InitialValue=throttle_hover  VectorParams1D=off  ShowAdditionalParam=off  OutDataTypeStr=double
  throttle_in1 : DataStoreMemory  DataStoreName=throttle_in  ReadBeforeWriteMsg=warning  WriteAfterWriteMsg=warning  WriteAfterReadMsg=warning  InitialValue=throttle_in  VectorParams1D=off  ShowAdditionalParam=off  OutDataTypeStr=double
  throttle_lower1 : DataStoreMemory  DataStoreName=throttle_lower  ReadBeforeWriteMsg=warning  WriteAfterWriteMsg=warning  WriteAfterReadMsg=warning  InitialValue=throttle_lower  VectorParams1D=off  ShowAdditionalParam=off  OutDataTypeStr=double
  throttle_max1 : DataStoreMemory  DataStoreName=throttle_max  ReadBeforeWriteMsg=warning  WriteAfterWriteMsg=warning  WriteAfterReadMsg=warning  InitialValue=throttle_max  VectorParams1D=off  ShowAdditionalParam=off  OutDataTypeStr=double
  throttle_min1 : DataStoreMemory  DataStoreName=throttle_min  ReadBeforeWriteMsg=warning  WriteAfterWriteMsg=warning  WriteAfterReadMsg=warning  InitialValue=throttle_min  VectorParams1D=off  ShowAdditionalParam=off  OutDataTypeStr=double
  throttle_off_rate : DataStoreMemory  DataStoreName=throttle_off_rate  ReadBeforeWriteMsg=warning  WriteAfterWriteMsg=warning  WriteAfterReadMsg=warning  InitialValue=throttle_off_rate  VectorParams1D=off  ShowAdditionalParam=off  OutDataTypeStr=double
  throttle_rpy_mix1 : DataStoreMemory  DataStoreName=throttle_rpy_mix  ReadBeforeWriteMsg=warning  WriteAfterWriteMsg=warning  WriteAfterReadMsg=warning  InitialValue=throttle_rpy_mix  VectorParams1D=off  ShowAdditionalParam=off  OutDataTypeStr=double
  throttle_rpy_mix_desired1 : DataStoreMemory  DataStoreName=throttle_rpy_mix_desired  ReadBeforeWriteMsg=warning  WriteAfterWriteMsg=warning  WriteAfterReadMsg=warning  InitialValue=throttle_rpy_mix_desired  VectorParams1D=off  ShowAdditionalParam=off  OutDataTypeStr=double
  throttle_slewrate1 : DataStoreMemory  DataStoreName=throttle_slewrate  ReadBeforeWriteMsg=warning  WriteAfterWriteMsg=warning  WriteAfterReadMsg=warning  InitialValue=throttle_slewrate  VectorParams1D=off  ShowAdditionalParam=off  OutDataTypeStr=double
  throttle_thrust_max1 : DataStoreMemory  DataStoreName=throttle_thrust_max  ReadBeforeWriteMsg=warning  WriteAfterWriteMsg=warning  WriteAfterReadMsg=warning  InitialValue=throttle_thrust_max  VectorParams1D=off  ShowAdditionalParam=off  OutDataTypeStr=double
  throttle_upper1 : DataStoreMemory  DataStoreName=throttle_upper  ReadBeforeWriteMsg=warning  WriteAfterWriteMsg=warning  WriteAfterReadMsg=warning  InitialValue=throttle_upper  VectorParams1D=off  ShowAdditionalParam=off  OutDataTypeStr=double
  thrust_boost1 : DataStoreMemory  DataStoreName=thrust_boost  ReadBeforeWriteMsg=warning  WriteAfterWriteMsg=warning  WriteAfterReadMsg=warning  InitialValue=thrust_boost  VectorParams1D=off  ShowAdditionalParam=off  OutDataTypeStr=double
  thrust_boost_ratio1 : DataStoreMemory  DataStoreName=thrust_boost_ratio  ReadBeforeWriteMsg=warning  WriteAfterWriteMsg=warning  WriteAfterReadMsg=warning  InitialValue=thrust_boost_ratio  VectorParams1D=off  ShowAdditionalParam=off  OutDataTypeStr=double
  thrust_error_angle1 : DataStoreMemory  DataStoreName=thrust_error_angle  ReadBeforeWriteMsg=warning  WriteAfterWriteMsg=warning  WriteAfterReadMsg=warning  InitialValue=thrust_error_angle  VectorParams1D=off  ShowAdditionalParam=off  OutDataTypeStr=double
  thrust_rpyt_out1 : DataStoreMemory  DataStoreName=thrust_rpyt_out  ReadBeforeWriteMsg=warning  WriteAfterWriteMsg=warning  WriteAfterReadMsg=warning  InitialValue=thrust_rpyt_out  VectorParams1D=off  ShowAdditionalParam=off  OutDataTypeStr=double
  thrust_slew_time1 : DataStoreMemory  DataStoreName=thrust_slew_time  ReadBeforeWriteMsg=warning  WriteAfterWriteMsg=warning  WriteAfterReadMsg=warning  InitialValue=thrust_slew_time  VectorParams1D=off  ShowAdditionalParam=off  OutDataTypeStr=double
  timeConstant1 : DataStoreMemory  DataStoreName=timeConstant  ReadBeforeWriteMsg=warning  WriteAfterWriteMsg=warning  WriteAfterReadMsg=warning  InitialValue=timeConstant  VectorParams1D=off  ShowAdditionalParam=off  OutDataTypeStr=double
  use_desvel_ff_z1 : DataStoreMemory  DataStoreName=use_desvel_ff_z  ReadBeforeWriteMsg=warning  WriteAfterWriteMsg=warning  WriteAfterReadMsg=warning  InitialValue=use_desvel_ff_z  VectorParams1D=off  ShowAdditionalParam=off  OutDataTypeStr=double
  use_sqrt_controller1 : DataStoreMemory  DataStoreName=use_sqrt_controller  ReadBeforeWriteMsg=warning  WriteAfterWriteMsg=warning  WriteAfterReadMsg=warning  InitialValue=use_sqrt_controller  ShowAdditionalParam=off  OutDataTypeStr=double
  vdot_filter1 : DataStoreMemory  DataStoreName=vdot_filter  ReadBeforeWriteMsg=warning  WriteAfterWriteMsg=warning  WriteAfterReadMsg=warning  InitialValue=vdot_filter  ShowAdditionalParam=off  OutDataTypeStr=double
  vel_desired1 : DataStoreMemory  DataStoreName=vel_desired  ReadBeforeWriteMsg=warning  WriteAfterWriteMsg=warning  WriteAfterReadMsg=warning  InitialValue=vel_desired  VectorParams1D=off  ShowAdditionalParam=off  OutDataTypeStr=double
  vel_dot1 : DataStoreMemory  DataStoreName=vel_dot  ReadBeforeWriteMsg=warning  WriteAfterWriteMsg=warning  WriteAfterReadMsg=warning  InitialValue=vel_dot  VectorParams1D=off  ShowAdditionalParam=off  OutDataTypeStr=double
  vel_error1 : DataStoreMemory  DataStoreName=vel_error  ReadBeforeWriteMsg=warning  WriteAfterWriteMsg=warning  WriteAfterReadMsg=warning  InitialValue=vel_error  VectorParams1D=off  ShowAdditionalParam=off  OutDataTypeStr=double
  vel_error_input1 : DataStoreMemory  DataStoreName=vel_error_input  ReadBeforeWriteMsg=warning  WriteAfterWriteMsg=warning  WriteAfterReadMsg=warning  InitialValue=vel_error_input  VectorParams1D=off  ShowAdditionalParam=off  OutDataTypeStr=double
  vel_forward_gain1 : DataStoreMemory  DataStoreName=vel_forward_gain  ReadBeforeWriteMsg=warning  WriteAfterWriteMsg=warning  WriteAfterReadMsg=warning  InitialValue=vel_forward_gain  VectorParams1D=off  ShowAdditionalParam=off  OutDataTypeStr=double
  vel_forward_integrator : DataStoreMemory  DataStoreName=vel_forward_integrator  ReadBeforeWriteMsg=warning  WriteAfterWriteMsg=warning  WriteAfterReadMsg=warning  InitialValue=vel_forward_integrator  VectorParams1D=off  ShowAdditionalParam=off  OutDataTypeStr=double
  vel_forward_last_pct1 : DataStoreMemory  DataStoreName=vel_forward_last_pct  ReadBeforeWriteMsg=warning  WriteAfterWriteMsg=warning  WriteAfterReadMsg=warning  InitialValue=vel_forward_last_pct  VectorParams1D=off  ShowAdditionalParam=off  OutDataTypeStr=double
  vel_forward_min_pitch1 : DataStoreMemory  DataStoreName=vel_forward_min_pitch  ReadBeforeWriteMsg=warning  WriteAfterWriteMsg=warning  WriteAfterReadMsg=warning  InitialValue=vel_forward_min_pitch  VectorParams1D=off  ShowAdditionalParam=off  OutDataTypeStr=double
  vel_forward_tail_tilt_max1 : DataStoreMemory  DataStoreName=vel_forward_tail_tilt_max  ReadBeforeWriteMsg=warning  WriteAfterWriteMsg=warning  WriteAfterReadMsg=warning  InitialValue=vel_forward_tail_tilt_max  VectorParams1D=off  ShowAdditionalParam=off  OutDataTypeStr=double
  vel_last1 : DataStoreMemory  DataStoreName=vel_last  ReadBeforeWriteMsg=warning  WriteAfterWriteMsg=warning  WriteAfterReadMsg=warning  InitialValue=vel_last  VectorParams1D=off  ShowAdditionalParam=off  OutDataTypeStr=double
  vel_target1 : DataStoreMemory  DataStoreName=vel_target  ReadBeforeWriteMsg=warning  WriteAfterWriteMsg=warning  WriteAfterReadMsg=warning  InitialValue=vel_target  VectorParams1D=off  ShowAdditionalParam=off  OutDataTypeStr=double
  vertAccLim1 : DataStoreMemory  DataStoreName=vertAccLim  ReadBeforeWriteMsg=warning  WriteAfterWriteMsg=warning  WriteAfterReadMsg=warning  InitialValue=vertAccLim  VectorParams1D=off  ShowAdditionalParam=off  OutDataTypeStr=double
  weathervane_gain1 : DataStoreMemory  DataStoreName=weathervane_gain  ReadBeforeWriteMsg=warning  WriteAfterWriteMsg=warning  WriteAfterReadMsg=warning  InitialValue=weathervane_gain  VectorParams1D=off  ShowAdditionalParam=off  OutDataTypeStr=double
  weathervane_last_output1 : DataStoreMemory  DataStoreName=weathervane_last_output  ReadBeforeWriteMsg=warning  WriteAfterWriteMsg=warning  WriteAfterReadMsg=warning  InitialValue=weathervane_last_output  VectorParams1D=off  ShowAdditionalParam=off  OutDataTypeStr=double
  weathervane_min_roll1 : DataStoreMemory  DataStoreName=weathervane_min_roll  ReadBeforeWriteMsg=warning  WriteAfterWriteMsg=warning  WriteAfterReadMsg=warning  InitialValue=weathervane_min_roll  VectorParams1D=off  ShowAdditionalParam=off  OutDataTypeStr=double
  yaw1 : DataStoreMemory  DataStoreName=yaw  ReadBeforeWriteMsg=warning  WriteAfterWriteMsg=warning  WriteAfterReadMsg=warning  InitialValue=yaw  VectorParams1D=off  ShowAdditionalParam=off  OutDataTypeStr=double
  yaw_factor1 : DataStoreMemory  DataStoreName=yaw_factor  ReadBeforeWriteMsg=warning  WriteAfterWriteMsg=warning  WriteAfterReadMsg=warning  InitialValue=yaw_factor  VectorParams1D=off  ShowAdditionalParam=off  OutDataTypeStr=double
  yaw_headroom1 : DataStoreMemory  DataStoreName=yaw_headroom  ReadBeforeWriteMsg=warning  WriteAfterWriteMsg=warning  WriteAfterReadMsg=warning  InitialValue=yaw_headroom  VectorParams1D=off  ShowAdditionalParam=off  OutDataTypeStr=double
  yaw_in1 : DataStoreMemory  DataStoreName=yaw_in  ReadBeforeWriteMsg=warning  WriteAfterWriteMsg=warning  WriteAfterReadMsg=warning  InitialValue=yaw_in  VectorParams1D=off  ShowAdditionalParam=off  OutDataTypeStr=double
  yaw_in_max : DataStoreMemory  DataStoreName=yaw_in_max  ReadBeforeWriteMsg=warning  WriteAfterWriteMsg=warning  WriteAfterReadMsg=warning  InitialValue=yaw_in_max  VectorParams1D=off  ShowAdditionalParam=off  OutDataTypeStr=double
  yaw_max_c2p1 : DataStoreMemory  DataStoreName=yaw_max_c2p  ReadBeforeWriteMsg=warning  WriteAfterWriteMsg=warning  WriteAfterReadMsg=warning  InitialValue=yaw_max_c2p  VectorParams1D=off  ShowAdditionalParam=off  OutDataTypeStr=double
  yaw_rate_max1 : DataStoreMemory  DataStoreName=yaw_rate_max  ReadBeforeWriteMsg=warning  WriteAfterWriteMsg=warning  WriteAfterReadMsg=warning  InitialValue=yaw_rate_max  VectorParams1D=off  ShowAdditionalParam=off  OutDataTypeStr=double
  z_accel_meas1 : DataStoreMemory  DataStoreName=z_accel_meas  ReadBeforeWriteMsg=warning  WriteAfterWriteMsg=warning  WriteAfterReadMsg=warning  InitialValue=z_accel_meas  VectorParams1D=off  ShowAdditionalParam=off  OutDataTypeStr=double
